simulink model "GridN1"  (R2021a)
settings: Solver=VariableStepAuto  StartTime=0.0  StopTime=1  FixedStep=1e-10  RelTol=1e-3
libraries: spsDistributedParametersLineLib x45, spsThreePhaseSeriesRLCLoadLib x20, spsThreePhaseVIMeasurementLib x3, spsGroundLib x1, spsThreePhaseSourceLib x1, spsSeriesRLCBranchLib x1, spspowerguiLib x1
settings Model: Creator=miair  LastModifiedBy=Admin
settings SolverCC: AlgebraicLoopSolver=TrustRegion
settings DataIOCC: ReturnWorkspaceOutputs=off
settings DebuggingCC: SFMachineParentedDataDiag=warning  ArithmeticOperatorsInVariantConditions=warning
settings SFSimCC: SimUseLocalCustomCode=off  CustomCodeUndefinedFunction=UseInterfaceOnly
settings RTWCC: RTWUseLocalCustomCode=off
settings CodeAppCC: StateflowObjectComments=on
settings SimscapeCC: SimscapeNormalizeSystem=off

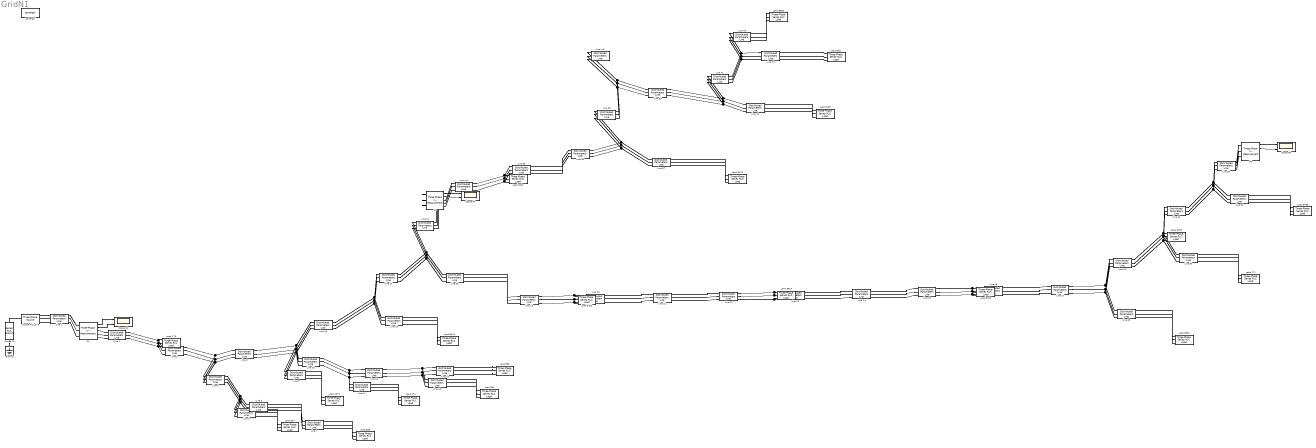
== system GridN1 ==
  Ground : spsGroundLib/Ground  LConnTagsString=a
  Line 1 : spsDistributedParametersLineLib/Distributed Parameters Line  Phases=3  Length=0.01  Frequency=50  Resistance=[0.476003738225748 0.351747138225748 0.351747138225748;0.351747138225748 0.476003738225748 0.351747138225748;0.351747138225748 0.351747138225748 0.476003738225748]  Inductance=[0.000705954362986426 0.000459934243504405 0.000459934243504405;0.000459934243504405 0.000705954362986426 0.000459934243504405;0.000459934243504405 0.000459934243504405 0.000705954362986426]  Capacitance=[5.7561313269996e-07 -1.37543883484145e-07 -1.37543912800485e-07;-1.37543883484145e-07 5.75613027339387e-07 -1.37543875208088e-07;-1.37543912800485e-07 -1.37543875208088e-07 5.75613005057695e-07]  x1=[0.0135819851168218 6580.60780006136 6580.6182267289;314.159265358979 314.159265358979 314.159265358979;-0.926204081652274 -0.816756558113271 -2.38755380781111]  x2=[0.0137023481415946 6580.57590971446 6580.58635696497;314.159265358979 314.159265358979 314.159265358979;-0.934430302579672 -0.816757783153402 -2.38755503539598]  x3=[0.0128763749933069 332.939719946223 332.945796056873;314.159265358979 314.159265358979 314.159265358979;-2.07623123292733 -0.796255794413397 -2.36710494899868]  x4=[0.0127279522499466 375.758691230381 375.75302064917;314.159265358979 314.159265358979 314.159265358979;1.03880908557987 -0.834961314041496 -2.40571318285691]  x5=2.2104317621921e-07  V1=[0.01488 9985 9985;314.2 314.2 314.2;0.4891 -0.0989 -1.67]  V2=[0.01499 9985 9985;314.2 314.2 314.2;0.4801 -0.0989 -1.67]  I1=[0.01357 505.2 505.2;314.2 314.2 314.2;-0.7953 -0.07837 -1.649]  I2=[0.01346 570.2 570.2;314.2 314.2 314.2;2.317 -0.1171 -1.688]  nHarmo=1  Measurements=None  Decoupling=off  VsMag0=0  VrMag0=0  VsAngle0=0  VrAngle0=0  IsMag0=0  IrMag0=0  IsAngle0=0  IrAngle0=0
      settings: SourceProductBaseCode=PS
  Line 10 : spsDistributedParametersLineLib/Distributed Parameters Line  Phases=3  Length=0.16  Frequency=50  Resistance=[0.646656091154803 0.0486237908083191 0.0486712220507153;0.0486237908083191 0.646561225344642 0.0486237934466192;0.0486712220507153 0.0486237934466192 0.646656091154803]  Inductance=[0.00282448912315926 0.00133270803418135 0.00132951476746136;0.00133270803418135 0.00282479813276775 0.00133799988507366;0.00132951476746136 0.00133799988507366 0.00282448912315926]  Capacitance=[7.89543174552926e-09 -1.85986777702161e-09 -1.7901190036642e-09;-1.85986777702161e-09 7.82540023894543e-09 -1.8957321828871e-09;-1.7901190036642e-09 -1.8957321828871e-09 7.91264394645417e-09]  x1=[85.9944639712659 6546.93050475178 6546.44352092211;314.159265358979 314.159265358979 314.159265358979;0.297132510613398 -0.901407935041179 -2.47234114362476]  x2=[85.9964448785897 6546.65446589105 6546.16802554073;314.159265358979 314.159265358979 314.159265358979;0.297142047123019 -0.901418200609058 -2.47235127057814]  x3=[0.0804619526636368 14.5654071899657 14.6911796185752;314.159265358979 314.159265358979 314.159265358979;0.235078954953871 -0.835037872721124 -2.40660973507596]  x4=[0.0702350961721193 18.8073119716894 18.934319702301;314.159265358979 314.159265358979 314.159265358979;0.367987664701655 -0.952972217807643 -2.52350664948334]  x5=7.66635634017784e-07  V1=[130.5 9934 9933;314.2 314.2 314.2;1.015 -0.1836 -1.754]  V2=[130.5 9933 9933;314.2 314.2 314.2;1.015 -0.1836 -1.754]  I1=[0.1221 22.1 22.29;314.2 314.2 314.2;0.9534 -0.1172 -1.689]  I2=[0.1066 28.54 28.73;314.2 314.2 314.2;1.086 -0.2351 -1.806]  nHarmo=1  Measurements=None  Decoupling=off  VsMag0=0  VrMag0=0  VsAngle0=0  VrAngle0=0  IsMag0=0  IrMag0=0  IsAngle0=0  IrAngle0=0
      settings: SourceProductBaseCode=PS
  Line 11 : spsDistributedParametersLineLib/Distributed Parameters Line  Phases=3  Length=0.16  Frequency=50  Resistance=[0.646656091154803 0.0486237908083191 0.0486712220507153;0.0486237908083191 0.646561225344642 0.0486237934466192;0.0486712220507153 0.0486237934466192 0.646656091154803]  Inductance=[0.00282448912315926 0.00133270803418135 0.00132951476746136;0.00133270803418135 0.00282479813276775 0.00133799988507366;0.00132951476746136 0.00133799988507366 0.00282448912315926]  Capacitance=[7.89543174552926e-09 -1.85986777702161e-09 -1.7901190036642e-09;-1.85986777702161e-09 7.82540023894543e-09 -1.8957321828871e-09;-1.7901190036642e-09 -1.8957321828871e-09 7.91264394645417e-09]  x1=[85.9964448785897 6546.65446589105 6546.16802554073;314.159265358979 314.159265358979 314.159265358979;0.297142047123019 -0.901418200609058 -2.47235127057814]  x2=[85.9976584945911 6546.47413610085 6545.98803986244;314.159265358979 314.159265358979 314.159265358979;0.297148477688424 -0.901424241770337 -2.47235721789357]  x3=[0.0785355624578365 15.3056638554528 15.4318437577526;314.159265358979 314.159265358979 314.159265358979;0.259013030174006 -0.858371763028016 -2.42967864630558]  x4=[0.0719518400150709 18.0351581181147 18.1620865019816;314.159265358979 314.159265358979 314.159265358979;0.338516704500895 -0.938129134970429 -2.50878862058241]  x5=7.66635634017784e-07  V1=[130.5 9933 9933;314.2 314.2 314.2;1.015 -0.1836 -1.754]  V2=[130.5 9933 9933;314.2 314.2 314.2;1.015 -0.1836 -1.755]  I1=[0.1192 23.22 23.42;314.2 314.2 314.2;0.9773 -0.1405 -1.712]  I2=[0.1092 27.37 27.56;314.2 314.2 314.2;1.057 -0.2203 -1.791]  nHarmo=1  Measurements=None  Decoupling=off  VsMag0=0  VrMag0=0  VsAngle0=0  VrAngle0=0  IsMag0=0  IrMag0=0  IsAngle0=0  IrAngle0=0
      settings: SourceProductBaseCode=PS
  Line 12 : spsDistributedParametersLineLib/Distributed Parameters Line  Phases=3  Length=0.18  Frequency=50  Resistance=[0.646656091154803 0.0486237908083191 0.0486712220507153;0.0486237908083191 0.646561225344642 0.0486237934466192;0.0486712220507153 0.0486237934466192 0.646656091154803]  Inductance=[0.00282448912315926 0.00133270803418135 0.00132951476746136;0.00133270803418135 0.00282479813276775 0.00133799988507366;0.00132951476746136 0.00133799988507366 0.00282448912315926]  Capacitance=[7.89543174552926e-09 -1.85986777702161e-09 -1.7901190036642e-09;-1.85986777702161e-09 7.82540023894543e-09 -1.8957321828871e-09;-1.7901190036642e-09 -1.8957321828871e-09 7.91264394645417e-09]  x1=[85.9964448785897 6546.65446589105 6546.16802554073;314.159265358979 314.159265358979 314.159265358979;0.297111941412071 -0.901442117619123 -2.47237521035551]  x2=[85.9972993196457 6546.54637248643 6546.06015563724;314.159265358979 314.159265358979 314.159265358979;0.297115479187386 -0.901446788951277 -2.47237983061846]  x3=[0.0770387830362932 15.9012798359736 16.0277069156014;314.159265358979 314.159265358979 314.159265358979;0.271434826795543 -0.88191367645825 -2.45304200019236]  x4=[0.0733797001123517 17.4185010889173 17.5453298819302;314.159265358979 314.159265358979 314.159265358979;0.323795655893711 -0.919479721591919 -2.49024653991903]  x5=8.62465088270006e-07  V1=[130.5 9933 9933;314.2 314.2 314.2;1.015 -0.1836 -1.755]  V2=[130.5 9933 9933;314.2 314.2 314.2;1.015 -0.1836 -1.755]  I1=[0.1169 24.13 24.32;314.2 314.2 314.2;0.9898 -0.1641 -1.735]  I2=[0.1114 26.43 26.62;314.2 314.2 314.2;1.042 -0.2016 -1.772]  nHarmo=1  Measurements=None  Decoupling=off  VsMag0=0  VrMag0=0  VsAngle0=0  VrAngle0=0  IsMag0=0  IrMag0=0  IsAngle0=0  IrAngle0=0
      settings: SourceProductBaseCode=PS
  Line 13 : spsDistributedParametersLineLib/Distributed Parameters Line  Phases=3  Length=0.53  Frequency=50  Resistance=[0.646656091154803 0.0486237908083191 0.0486712220507153;0.0486237908083191 0.646561225344642 0.0486237934466192;0.0486712220507153 0.0486237934466192 0.646656091154803]  Inductance=[0.00282448912315926 0.00133270803418135 0.00132951476746136;0.00133270803418135 0.00282479813276775 0.00133799988507366;0.00132951476746136 0.00133799988507366 0.00282448912315926]  Capacitance=[7.89543174552926e-09 -1.85986777702161e-09 -1.7901190036642e-09;-1.85986777702161e-09 7.82540023894543e-09 -1.8957321828871e-09;-1.7901190036642e-09 -1.8957321828871e-09 7.91264394645417e-09]  x1=[85.9972993196455 6546.54637248643 6546.06015563724;314.159265358979 314.159265358979 314.159265358979;0.296588629245806 -0.901865336627409 -2.47279877672234]  x2=[85.999109686468 6546.2820331029 6545.79632491974;314.159265358979 314.159265358979 314.159265358979;0.296597976971236 -0.901874451699163 -2.47280775550619]  x3=[0.0766475627213019 16.0457568642052 16.1721358047216;314.159265358979 314.159265358979 314.159265358979;0.278553064422003 -0.884195825609553 -2.45528139945166]  x4=[0.0737204509155215 17.2589219147414 17.3856160487695;314.159265358979 314.159265358979 314.159265358979;0.3145362068788 -0.918913142041838 -2.4897144121643]  x5=2.53948053768391e-06  V1=[130.5 9933 9933;314.2 314.2 314.2;1.015 -0.184 -1.755]  V2=[130.5 9933 9932;314.2 314.2 314.2;1.015 -0.184 -1.755]  I1=[0.1163 24.35 24.54;314.2 314.2 314.2;0.9969 -0.1663 -1.737]  I2=[0.1119 26.19 26.38;314.2 314.2 314.2;1.033 -0.2011 -1.772]  nHarmo=1  Measurements=None  Decoupling=off  VsMag0=0  VrMag0=0  VsAngle0=0  VrAngle0=0  IsMag0=0  IrMag0=0  IsAngle0=0  IrAngle0=0
      settings: SourceProductBaseCode=PS
  Line 14 : spsDistributedParametersLineLib/Distributed Parameters Line  Phases=3  Length=2.16  Frequency=50  Resistance=[0.646656091154803 0.0486237908083191 0.0486712220507153;0.0486237908083191 0.646561225344642 0.0486237934466192;0.0486712220507153 0.0486237934466192 0.646656091154803]  Inductance=[0.00282448912315926 0.00133270803418135 0.00132951476746136;0.00133270803418135 0.00282479813276775 0.00133799988507366;0.00132951476746136 0.00133799988507366 0.00282448912315926]  Capacitance=[7.89543174552926e-09 -1.85986777702161e-09 -1.7901190036642e-09;-1.85986777702161e-09 7.82540023894543e-09 -1.8957321828871e-09;-1.7901190036642e-09 -1.8957321828871e-09 7.91264394645417e-09]  x1=[85.9972993196455 6546.54637248643 6546.06015563724;314.159265358979 314.159265358979 314.159265358979;0.294135013803574 -0.903814572947683 -2.47474986857757]  x2=[85.9995705439625 6546.29754411503 6545.81188305122;314.159265358979 314.159265358979 314.159265358979;0.29414239813252 -0.90382784404018 -2.47476303451906]  x3=[0.0754794263753424 16.467720066683 16.5937728872859;314.159265358979 314.159265358979 314.159265358979;0.286520713788774 -0.901964753453352 -2.47293834107752]  x4=[0.0747483168592489 16.7703048358143 16.8964299339934;314.159265358979 314.159265358979 314.159265358979;0.298562747055325 -0.908206004743712 -2.47910645537711]  x5=1.03495810592401e-05  V1=[130.5 9933 9933;314.2 314.2 314.2;1.012 -0.186 -1.757]  V2=[130.5 9933 9932;314.2 314.2 314.2;1.012 -0.186 -1.757]  I1=[0.1145 24.99 25.18;314.2 314.2 314.2;1.005 -0.1841 -1.755]  I2=[0.1134 25.45 25.64;314.2 314.2 314.2;1.017 -0.1904 -1.761]  nHarmo=1  Measurements=None  Decoupling=off  VsMag0=0  VrMag0=0  VsAngle0=0  VrAngle0=0  IsMag0=0  IrMag0=0  IsAngle0=0  IrAngle0=0
      settings: SourceProductBaseCode=PS
  Line 15 : spsDistributedParametersLineLib/Distributed Parameters Line  Phases=3  Length=4.06  Frequency=50  Resistance=[0.502970710632245 0.0486237908083191 0.0486712220507153;0.0486237908083191 0.502875844822084 0.0486237934466192;0.0486712220507153 0.0486237934466192 0.502970710632245]  Inductance=[0.00286900545038753 0.00133270803418135 0.00132951476746136;0.00133270803418135 0.00286931445999602 0.00133799988507366;0.00132951476746136 0.00133799988507366 0.00286900545038753]  Capacitance=[8.11484299003193e-09 -1.94249816214699e-09 -1.86930692621136e-09;-1.94249816214699e-09 8.0425699231653e-09 -1.98049571960044e-09;-1.86930692621136e-09 -1.98049571960044e-09 8.13337738722527e-09]  x1=[155.130058091746 6546.90392964469 6546.32991141257;314.159265358979 314.159265358979 314.159265358979;0.274010343197794 -0.899988695828293 -2.47095312062203]  x2=[155.136487397732 6511.09041009802 6510.62379376133;314.159265358979 314.159265358979 314.159265358979;0.272333769665952 -0.903385149921619 -2.47432401319414]  x3=[0.10391403445318 4.32286136277482 4.3539078763867;314.159265358979 314.159265358979 314.159265358979;0.152577548487083 0.302540110540726 -1.29846084646846]  x4=[0.168935784291522 31.8497990242347 31.9649152376635;314.159265358979 314.159265358979 314.159265358979;0.342256765474295 -1.03135915522522 -2.60124142850109]  x5=1.96604952826627e-05  V1=[235.4 9934 9933;314.2 314.2 314.2;0.9921 -0.1821 -1.753]  V2=[235.4 9879 9879;314.2 314.2 314.2;0.9908 -0.1855 -1.756]  I1=[0.1683 6.565 6.576;314.2 314.2 314.2;0.8807 1.024 -0.5817]  I2=[0.2456 48.35 48.5;314.2 314.2 314.2;1.062 -0.3137 -1.883]  nHarmo=1  Measurements=None  Decoupling=off  VsMag0=0  VrMag0=0  VsAngle0=0  VrAngle0=0  IsMag0=0  IrMag0=0  IsAngle0=0  IrAngle0=0
      settings: SourceProductBaseCode=PS
  Line 16 : spsDistributedParametersLineLib/Distributed Parameters Line  Phases=3  Length=0.01  Frequency=50  Resistance=[0.646656091154803 0.0486237908083191 0.0486712220507153;0.0486237908083191 0.646561225344642 0.0486237934466192;0.0486712220507153 0.0486237934466192 0.646656091154803]  Inductance=[0.00282448912315926 0.00133270803418135 0.00132951476746136;0.00133270803418135 0.00282479813276775 0.00133799988507366;0.00132951476746136 0.00133799988507366 0.00282448912315926]  Capacitance=[7.89543174552926e-09 -1.85986777702161e-09 -1.7901190036642e-09;-1.85986777702161e-09 7.82540023894543e-09 -1.8957321828871e-09;-1.7901190036642e-09 -1.8957321828871e-09 7.91264394645417e-09]  x1=[86.3836277831307 6511.11801645557 6510.73918186067;314.159265358979 314.159265358979 314.159265358979;0.296859447111635 -0.904624882143572 -2.4755324376731]  x2=[86.3836330279052 6511.11723795004 6510.73840482828;314.159265358979 314.159265358979 314.159265358979;0.296859474579558 -0.904624908354452 -2.47553246347659]  x3=[0.075755124590947 16.4755952702995 16.6018616731868;314.159265358979 314.159265358979 314.159265358979;0.294122728550855 -0.901862047196781 -2.4727919470391]  x4=[0.075301162455798 16.6643113475344 16.7906304355618;314.159265358979 314.159265358979 314.159265358979;0.299597594398029 -0.907368346005886 -2.47825404656015]  x5=4.79147271261115e-08  V1=[131.1 9879 9879;314.2 314.2 314.2;1.016 -0.1868 -1.758]  V2=[131.1 9879 9879;314.2 314.2 314.2;1.016 -0.1868 -1.758]  I1=[0.115 25 25.19;314.2 314.2 314.2;1.013 -0.184 -1.755]  I2=[0.1143 25.29 25.48;314.2 314.2 314.2;1.019 -0.1895 -1.76]  nHarmo=1  Measurements=None  Decoupling=off  VsMag0=0  VrMag0=0  VsAngle0=0  VrAngle0=0  IsMag0=0  IrMag0=0  IsAngle0=0  IrAngle0=0
      settings: SourceProductBaseCode=PS
  Line 17 : spsDistributedParametersLineLib/Distributed Parameters Line  Phases=3  Length=0.35  Frequency=50  Resistance=[0.646656091154803 0.0486237908083191 0.0486712220507153;0.0486237908083191 0.646561225344642 0.0486237934466192;0.0486712220507153 0.0486237934466192 0.646656091154803]  Inductance=[0.00282448912315926 0.00133270803418135 0.00132951476746136;0.00133270803418135 0.00282479813276775 0.00133799988507366;0.00132951476746136 0.00133799988507366 0.00282448912315926]  Capacitance=[7.89543174552926e-09 -1.85986777702161e-09 -1.7901190036642e-09;-1.85986777702161e-09 7.82540023894543e-09 -1.8957321828871e-09;-1.7901190036642e-09 -1.8957321828871e-09 7.91264394645417e-09]  x1=[86.3836277831307 6511.11801645557 6510.73918186067;314.159265358979 314.159265358979 314.159265358979;0.296347650025526 -0.905031471314672 -2.4759394138883]  x2=[86.4097152949425 6507.31425320866 6506.94452871459;314.159265358979 314.159265358979 314.159265358979;0.296462312233359 -0.905281202958687 -2.4761870329915]  x3=[0.109465414980559 4.31753359742384 4.35145979089518;314.159265358979 314.159265358979 314.159265358979;0.0135914404706076 0.296780704754496 -1.30398448333316]  x4=[0.0551442407666985 31.8173296486231 31.9338693613861;314.159265358979 314.159265358979 314.159265358979;0.882642018156363 -1.03228675249212 -2.60219232773787]  x5=1.6770154494139e-06  V1=[131.1 9879 9879;314.2 314.2 314.2;1.015 -0.1872 -1.758]  V2=[131.2 9874 9873;314.2 314.2 314.2;1.015 -0.1874 -1.758]  I1=[0.1764 6.557 6.572;314.2 314.2 314.2;0.7506 1.018 -0.5873]  I2=[0.07492 48.3 48.46;314.2 314.2 314.2;1.678 -0.3147 -1.884]  nHarmo=1  Measurements=None  Decoupling=off  VsMag0=0  VrMag0=0  VsAngle0=0  VrAngle0=0  IsMag0=0  IrMag0=0  IsAngle0=0  IrAngle0=0
      settings: SourceProductBaseCode=PS
  Line 18 : spsDistributedParametersLineLib/Distributed Parameters Line  Phases=3  Length=0.26  Frequency=50  Resistance=[0.646656091154803 0.0486237908083191 0.0486712220507153;0.0486237908083191 0.646561225344642 0.0486237934466192;0.0486712220507153 0.0486237934466192 0.646656091154803]  Inductance=[0.00282448912315926 0.00133270803418135 0.00132951476746136;0.00133270803418135 0.00282479813276775 0.00133799988507366;0.00132951476746136 0.00133799988507366 0.00282448912315926]  Capacitance=[7.89543174552926e-09 -1.85986777702161e-09 -1.7901190036642e-09;-1.85986777702161e-09 7.82540023894543e-09 -1.8957321828871e-09;-1.7901190036642e-09 -1.8957321828871e-09 7.91264394645417e-09]  x1=[86.4097152949424 6507.31425320866 6506.94452871459;314.159265358979 314.159265358979 314.159265358979;0.296597787932625 -0.905173576413396 -2.47607930399336]  x2=[86.4164234767737 6506.31319209991 6505.94386622124;314.159265358979 314.159265358979 314.159265358979;0.296676077842439 -0.90529675193356 -2.47620177288688]  x3=[0.0940058289360008 10.0710803597759 10.1963204188777;314.159265358979 314.159265358979 314.159265358979;0.220423677789878 -0.911182921321596 -2.48235367189124]  x4=[0.0577970860777915 23.0375917576632 23.1647009597948;314.159265358979 314.159265358979 314.159265358979;0.420279554992001 -0.902858499466097 -2.47362985744283]  x5=1.2457829052789e-06  V1=[131.2 9874 9873;314.2 314.2 314.2;1.016 -0.1873 -1.758]  V2=[131.2 9872 9872;314.2 314.2 314.2;1.016 -0.1874 -1.758]  I1=[0.1427 15.28 15.47;314.2 314.2 314.2;0.9392 -0.1933 -1.765]  I2=[0.08773 34.96 35.15;314.2 314.2 314.2;1.14 -0.185 -1.756]  nHarmo=1  Measurements=None  Decoupling=off  VsMag0=0  VrMag0=0  VsAngle0=0  VrAngle0=0  IsMag0=0  IrMag0=0  IsAngle0=0  IrAngle0=0
      settings: SourceProductBaseCode=PS
  Line 19 : spsDistributedParametersLineLib/Distributed Parameters Line  Phases=3  Length=0.03  Frequency=50  Resistance=[0.476003738225748 0.351747138225748 0.351747138225748;0.351747138225748 0.476003738225748 0.351747138225748;0.351747138225748 0.351747138225748 0.476003738225748]  Inductance=[0.000705954362986426 0.000459934243504405 0.000459934243504405;0.000459934243504405 0.000705954362986426 0.000459934243504405;0.000459934243504405 0.000459934243504405 0.000705954362986426]  Capacitance=[5.7561313269996e-07 -1.37543883484145e-07 -1.37543912800485e-07;-1.37543883484145e-07 5.75613027339387e-07 -1.37543875208088e-07;-1.37543912800485e-07 -1.37543875208088e-07 5.75613005057695e-07]  x1=[1.80349077964358 6506.96689280743 6507.23152701917;314.159265358979 314.159265358979 314.159265358979;0.568507403599857 -0.823462772990433 -2.39421460640899]  x2=[1.80349908463451 6506.94280065842 6507.20743625873;314.159265358979 314.159265358979 314.159265358979;0.568466669705737 -0.823465104058031 -2.39421693847239]  x3=[0.0240219359496491 343.799843304301 343.813477118347;314.159265358979 314.159265358979 314.159265358979;0.492004045456063 -0.823628998476846 -2.39438530592288]  x4=[0.0251371408204683 356.767166807137 356.781970901396;314.159265358979 314.159265358979 314.159265358979;0.641366971008245 -0.823427454004275 -2.39417497717186]  x5=6.63129528657629e-07  V1=[2.826 9873 9874;314.2 314.2 314.2;1.332 -0.1056 -1.676]  V2=[2.826 9873 9874;314.2 314.2 314.2;1.332 -0.1056 -1.676]  I1=[0.03756 521.7 521.7;314.2 314.2 314.2;1.259 -0.1058 -1.677]  I2=[0.03945 541.3 541.4;314.2 314.2 314.2;1.402 -0.1056 -1.676]  nHarmo=1  Measurements=None  Decoupling=off  VsMag0=0  VrMag0=0  VsAngle0=0  VrAngle0=0  IsMag0=0  IrMag0=0  IsAngle0=0  IrAngle0=0
      settings: SourceProductBaseCode=PS
  Line 2 : spsDistributedParametersLineLib/Distributed Parameters Line  Phases=3  Length=0.67  Frequency=50  Resistance=[0.502970710632245 0.0486237908083191 0.0486712220507153;0.0486237908083191 0.502875844822084 0.0486237934466192;0.0486712220507153 0.0486237934466192 0.502970710632245]  Inductance=[0.00286900545038753 0.00133270803418135 0.00132951476746136;0.00133270803418135 0.00286931445999602 0.00133799988507366;0.00132951476746136 0.00133799988507366 0.00286900545038753]  Capacitance=[8.11484299003193e-09 -1.94249816214699e-09 -1.86930692621136e-09;-1.94249816214699e-09 8.0425699231653e-09 -1.98049571960044e-09;-1.86930692621136e-09 -1.98049571960044e-09 8.13337738722527e-09]  x1=[155.130864966467 6579.86288650135 6579.19403824536;314.159265358979 314.159265358979 314.159265358979;0.280572916473346 -0.892956956254344 -2.46393908894624]  x2=[155.129993894483 6571.12588097019 6570.48183439309;314.159265358979 314.159265358979 314.159265358979;0.280210089543806 -0.893696316191029 -2.46467257592617]  x3=[0.0936269338507397 8.28080195745267 8.1875967056366;314.159265358979 314.159265358979 314.159265358979;0.126927443731738 1.27624388214372 -0.306383861829034]  x4=[0.180082285305984 38.7443835177047 38.8603787264615;314.159265358979 314.159265358979 314.159265358979;0.359177992222435 -1.07116495488925 -2.64099140895834]  x5=3.24446597029163e-06  V1=[235.4 9984 9983;314.2 314.2 314.2;0.9985 -0.1751 -1.746]  V2=[235.4 9971 9970;314.2 314.2 314.2;0.9982 -0.1758 -1.747]  I1=[0.1527 12.59 12.4;314.2 314.2 314.2;0.8579 1.995 0.4132]  I2=[0.2625 58.81 58.96;314.2 314.2 314.2;1.079 -0.3535 -1.923]  nHarmo=1  Measurements=None  Decoupling=off  VsMag0=0  VrMag0=0  VsAngle0=0  VrAngle0=0  IsMag0=0  IrMag0=0  IsAngle0=0  IrAngle0=0
      settings: SourceProductBaseCode=PS
  Line 20 : spsDistributedParametersLineLib/Distributed Parameters Line  Phases=3  Length=0.06  Frequency=50  Resistance=[0.476003738225748 0.351747138225748 0.351747138225748;0.351747138225748 0.476003738225748 0.351747138225748;0.351747138225748 0.351747138225748 0.476003738225748]  Inductance=[0.000705954362986426 0.000459934243504405 0.000459934243504405;0.000459934243504405 0.000705954362986426 0.000459934243504405;0.000459934243504405 0.000459934243504405 0.000705954362986426]  Capacitance=[5.7561313269996e-07 -1.37543883484145e-07 -1.37543912800485e-07;-1.37543883484145e-07 5.75613027339387e-07 -1.37543875208088e-07;-1.37543912800485e-07 -1.37543875208088e-07 5.75613005057695e-07]  x1=[1.80349908463435 6506.94280065843 6507.20743625873;314.159265358979 314.159265358979 314.159265358979;0.568258341420157 -0.823589942694024 -2.39434177709874]  x2=[1.80351546829951 6506.90345923597 6507.16809797319;314.159265358979 314.159265358979 314.159265358979;0.568177174345155 -0.823594380959789 -2.39434621735615]  x3=[0.0240130059935537 344.689458476285 344.70313048417;314.159265358979 314.159265358979 314.159265358979;0.491956343910604 -0.824953446673106 -2.39570974436397]  x4=[0.0251275086274899 355.769214247355 355.783979573751;314.159265358979 314.159265358979 314.159265358979;0.640683073045103 -0.822519085690189 -2.39326659996042]  x5=1.32625905731526e-06  V1=[2.826 9873 9874;314.2 314.2 314.2;1.332 -0.1057 -1.676]  V2=[2.826 9873 9874;314.2 314.2 314.2;1.332 -0.1057 -1.677]  I1=[0.03754 523 523;314.2 314.2 314.2;1.259 -0.1071 -1.678]  I2=[0.03944 539.8 539.9;314.2 314.2 314.2;1.401 -0.1047 -1.675]  nHarmo=1  Measurements=None  Decoupling=off  VsMag0=0  VrMag0=0  VsAngle0=0  VrAngle0=0  IsMag0=0  IrMag0=0  IsAngle0=0  IrAngle0=0
      settings: SourceProductBaseCode=PS
  Line 21 : spsDistributedParametersLineLib/Distributed Parameters Line  Phases=3  Length=0.2  Frequency=50  Resistance=[0.646656091154803 0.0486237908083191 0.0486712220507153;0.0486237908083191 0.646561225344642 0.0486237934466192;0.0486712220507153 0.0486237934466192 0.646656091154803]  Inductance=[0.00282448912315926 0.00133270803418135 0.00132951476746136;0.00133270803418135 0.00282479813276775 0.00133799988507366;0.00132951476746136 0.00133799988507366 0.00282448912315926]  Capacitance=[7.89543174552926e-09 -1.85986777702161e-09 -1.7901190036642e-09;-1.85986777702161e-09 7.82540023894543e-09 -1.8957321828871e-09;-1.7901190036642e-09 -1.8957321828871e-09 7.91264394645417e-09]  x1=[86.4156775370292 6506.24976374386 6505.88045131294;314.159265358979 314.159265358979 314.159265358979;0.296757442469757 -0.905231770339363 -2.47613672584176]  x2=[86.4198873770657 6505.62270406743 6505.25347886743;314.159265358979 314.159265358979 314.159265358979;0.296811157398845 -0.905318825738908 -2.47622331895673]  x3=[0.0915214048129825 11.0184276621565 11.1439055827763;314.159265358979 314.159265358979 314.159265358979;0.237528372241948 -0.939888068634841 -2.51068855775993]  x4=[0.0599840015892358 22.0976245780948 22.2245410295841;314.159265358979 314.159265358979 314.159265358979;0.38688459691695 -0.888198292322438 -2.45905890793362]  x5=9.5829454252223e-07  V1=[131.2 9872 9872;314.2 314.2 314.2;1.016 -0.1874 -1.758]  V2=[131.2 9871 9871;314.2 314.2 314.2;1.016 -0.1875 -1.758]  I1=[0.1389 16.72 16.91;314.2 314.2 314.2;0.9563 -0.222 -1.793]  I2=[0.09104 33.53 33.72;314.2 314.2 314.2;1.106 -0.1703 -1.741]  nHarmo=1  Measurements=None  Decoupling=off  VsMag0=0  VrMag0=0  VsAngle0=0  VrAngle0=0  IsMag0=0  IrMag0=0  IsAngle0=0  IrAngle0=0
      settings: SourceProductBaseCode=PS
  Line 22 : spsDistributedParametersLineLib/Distributed Parameters Line  Phases=3  Length=0.05  Frequency=50  Resistance=[0.476003738225748 0.351747138225748 0.351747138225748;0.351747138225748 0.476003738225748 0.351747138225748;0.351747138225748 0.351747138225748 0.476003738225748]  Inductance=[0.000705954362986426 0.000459934243504405 0.000459934243504405;0.000459934243504405 0.000705954362986426 0.000459934243504405;0.000459934243504405 0.000459934243504405 0.000705954362986426]  Capacitance=[5.7561313269996e-07 -1.37543883484145e-07 -1.37543912800485e-07;-1.37543883484145e-07 5.75613027339387e-07 -1.37543875208088e-07;-1.37543912800485e-07 -1.37543875208088e-07 5.75613005057695e-07]  x1=[1.81872127937186 6506.27610314953 6506.5412101485;314.159265358979 314.159265358979 314.159265358979;0.572739489358775 -0.823639824767842 -2.39439120314015]  x2=[1.81873407318244 6506.24299562844 6506.50810513395;314.159265358979 314.159265358979 314.159265358979;0.572673891127853 -0.823643443820417 -2.39439482381432]  x3=[0.0242231513539572 344.670879322376 344.68458384404;314.159265358979 314.159265358979 314.159265358979;0.498933104195823 -0.824739694137653 -2.39549543281646]  x4=[0.02532942018017 355.751316792513 355.766100937454;314.159265358979 314.159265358979 314.159265358979;0.642913048433806 -0.822782616536565 -2.39352977372954]  x5=1.10521588109605e-06  V1=[2.85 9872 9873;314.2 314.2 314.2;1.336 -0.1058 -1.677]  V2=[2.85 9872 9873;314.2 314.2 314.2;1.336 -0.1058 -1.677]  I1=[0.03787 523 523;314.2 314.2 314.2;1.265 -0.1069 -1.678]  I2=[0.03975 539.8 539.8;314.2 314.2 314.2;1.403 -0.1049 -1.676]  nHarmo=1  Measurements=None  Decoupling=off  VsMag0=0  VrMag0=0  VsAngle0=0  VrAngle0=0  IsMag0=0  IrMag0=0  IsAngle0=0  IrAngle0=0
      settings: SourceProductBaseCode=PS
  Line 23 : spsDistributedParametersLineLib/Distributed Parameters Line  Phases=3  Length=0.05  Frequency=50  Resistance=[0.476003738225748 0.351747138225748 0.351747138225748;0.351747138225748 0.476003738225748 0.351747138225748;0.351747138225748 0.351747138225748 0.476003738225748]  Inductance=[0.000705954362986426 0.000459934243504405 0.000459934243504405;0.000459934243504405 0.000705954362986426 0.000459934243504405;0.000459934243504405 0.000459934243504405 0.000705954362986426]  Capacitance=[5.7561313269996e-07 -1.37543883484145e-07 -1.37543912800485e-07;-1.37543883484145e-07 5.75613027339387e-07 -1.37543875208088e-07;-1.37543912800485e-07 -1.37543875208088e-07 5.75613005057695e-07]  x1=[1.81873407318247 6506.24299562844 6506.50810513395;314.159265358979 314.159265358979 314.159265358979;0.572673891127767 -0.823643443820417 -2.39439482381432]  x2=[1.81874665516727 6506.21722820899 6506.48234052024;314.159265358979 314.159265358979 314.159265358979;0.572608571318828 -0.823646869350555 -2.39439825096607]  x3=[0.0242227990722459 345.612328664751 345.626073424913;314.159265358979 314.159265358979 314.159265358979;0.499219322631955 -0.825850429726011 -2.39660615929487]  x4=[0.0253288933872046 354.807869311172 354.822616843042;314.159265358979 314.159265358979 314.159265358979;0.642511794453256 -0.82170242285628 -2.39244957127083]  x5=1.10521588109605e-06  V1=[2.85 9872 9873;314.2 314.2 314.2;1.336 -0.1058 -1.677]  V2=[2.85 9872 9873;314.2 314.2 314.2;1.336 -0.1058 -1.677]  I1=[0.03787 524.4 524.4;314.2 314.2 314.2;1.265 -0.108 -1.679]  I2=[0.03975 538.4 538.4;314.2 314.2 314.2;1.403 -0.1038 -1.675]  nHarmo=1  Measurements=None  Decoupling=off  VsMag0=0  VrMag0=0  VsAngle0=0  VrAngle0=0  IsMag0=0  IrMag0=0  IsAngle0=0  IrAngle0=0
      settings: SourceProductBaseCode=PS
  Line 24 : spsDistributedParametersLineLib/Distributed Parameters Line  Phases=3  Length=0.07  Frequency=50  Resistance=[0.646656091154803 0.0486237908083191 0.0486712220507153;0.0486237908083191 0.646561225344642 0.0486237934466192;0.0486712220507153 0.0486237934466192 0.646656091154803]  Inductance=[0.00282448912315926 0.00133270803418135 0.00132951476746136;0.00133270803418135 0.00282479813276775 0.00133799988507366;0.00132951476746136 0.00133799988507366 0.00282448912315926]  Capacitance=[7.89543174552926e-09 -1.85986777702161e-09 -1.7901190036642e-09;-1.85986777702161e-09 7.82540023894543e-09 -1.8957321828871e-09;-1.7901190036642e-09 -1.8957321828871e-09 7.91264394645417e-09]  x1=[86.4192070770427 6505.56383378223 6505.19462260516;314.159265358979 314.159265358979 314.159265358979;0.296997423813308 -0.905170409868426 -2.47607475819285]  x2=[86.4203532262805 6505.39397464631 6505.02472042426;314.159265358979 314.159265358979 314.159265358979;0.297013900777833 -0.90519809985593 -2.47610231497634]  x3=[0.0890553814813472 11.9746385535509 12.1002847514108;314.159265358979 314.159265358979 314.159265358979;0.255140561932488 -0.96277099212005 -2.53331866081606]  x4=[0.06224838038178 21.1652048696928 21.2919280563146;314.159265358979 314.159265358979 314.159265358979;0.356790003617149 -0.872681161888096 -2.44364213900161]  x5=3.3540308988278e-07  V1=[131.2 9871 9871;314.2 314.2 314.2;1.016 -0.1873 -1.758]  V2=[131.2 9871 9870;314.2 314.2 314.2;1.016 -0.1873 -1.758]  I1=[0.1352 18.17 18.36;314.2 314.2 314.2;0.9739 -0.2449 -1.815]  I2=[0.09448 32.11 32.31;314.2 314.2 314.2;1.076 -0.1548 -1.726]  nHarmo=1  Measurements=None  Decoupling=off  VsMag0=0  VrMag0=0  VsAngle0=0  VrAngle0=0  IsMag0=0  IrMag0=0  IsAngle0=0  IrAngle0=0
      settings: SourceProductBaseCode=PS
  Line 25 : spsDistributedParametersLineLib/Distributed Parameters Line  Phases=3  Length=0.28  Frequency=50  Resistance=[0.476003738225748 0.351747138225748 0.351747138225748;0.351747138225748 0.476003738225748 0.351747138225748;0.351747138225748 0.351747138225748 0.476003738225748]  Inductance=[0.000705954362986426 0.000459934243504405 0.000459934243504405;0.000459934243504405 0.000705954362986426 0.000459934243504405;0.000459934243504405 0.000459934243504405 0.000705954362986426]  Capacitance=[5.7561313269996e-07 -1.37543883484145e-07 -1.37543912800485e-07;-1.37543883484145e-07 5.75613027339387e-07 -1.37543875208088e-07;-1.37543912800485e-07 -1.37543875208088e-07 5.75613005057695e-07]  x1=[1.8230209208266 6506.04728504326 6506.31246540836;314.159265358979 314.159265358979 314.159265358979;0.572485854467426 -0.824631656746514 -2.39538290476063]  x2=[1.8230863268609 6505.89775727232 6506.16295295788;314.159265358979 314.159265358979 314.159265358979;0.572128374768087 -0.824649547749504 -2.39540080477212]  x3=[0.0242137936707559 345.201325872334 345.215060458315;314.159265358979 314.159265358979 314.159265358979;0.499985173074447 -0.826625035667704 -2.39738059969799]  x4=[0.0253117804131848 354.382690207975 354.397421274766;314.159265358979 314.159265358979 314.159265358979;0.639582549208556 -0.823858187108396 -2.39460524216789]  x5=6.18920893413787e-06  V1=[2.856 9872 9872;314.2 314.2 314.2;1.336 -0.1068 -1.678]  V2=[2.856 9872 9872;314.2 314.2 314.2;1.335 -0.1068 -1.678]  I1=[0.03786 523.8 523.8;314.2 314.2 314.2;1.266 -0.1088 -1.68]  I2=[0.03972 537.7 537.7;314.2 314.2 314.2;1.4 -0.106 -1.677]  nHarmo=1  Measurements=None  Decoupling=off  VsMag0=0  VrMag0=0  VsAngle0=0  VrAngle0=0  IsMag0=0  IrMag0=0  IsAngle0=0  IrAngle0=0
      settings: SourceProductBaseCode=PS
  Line 26 : spsDistributedParametersLineLib/Distributed Parameters Line  Phases=3  Length=0.28  Frequency=50  Resistance=[0.476003738225748 0.351747138225748 0.351747138225748;0.351747138225748 0.476003738225748 0.351747138225748;0.351747138225748 0.351747138225748 0.476003738225748]  Inductance=[0.000705954362986426 0.000459934243504405 0.000459934243504405;0.000459934243504405 0.000705954362986426 0.000459934243504405;0.000459934243504405 0.000459934243504405 0.000705954362986426]  Capacitance=[5.7561313269996e-07 -1.37543883484145e-07 -1.37543912800485e-07;-1.37543883484145e-07 5.75613027339387e-07 -1.37543875208088e-07;-1.37543912800485e-07 -1.37543875208088e-07 5.75613005057695e-07]  x1=[1.82308632686094 6505.89775727232 6506.16295295788;314.159265358979 314.159265358979 314.159265358979;0.572128374768 -0.824649547749504 -2.39540080477212]  x2=[1.82314506449276 6505.80768545556 6506.07289888839;314.159265358979 314.159265358979 314.159265358979;0.571779641739294 -0.82466414612788 -2.39541541215957]  x3=[0.0242118510820579 346.700996752661 346.714795023725;314.159265358979 314.159265358979 314.159265358979;0.501603433603007 -0.827563523571792 -2.39831907914342]  x4=[0.0253088324522552 352.871323867619 352.885995815209;314.159265358979 314.159265358979 314.159265358979;0.637346398018359 -0.822956511028876 -2.39370355757977]  x5=6.18920893413787e-06  V1=[2.856 9872 9872;314.2 314.2 314.2;1.335 -0.1068 -1.678]  V2=[2.856 9871 9872;314.2 314.2 314.2;1.335 -0.1068 -1.678]  I1=[0.03786 526.1 526.1;314.2 314.2 314.2;1.267 -0.1097 -1.68]  I2=[0.03971 535.4 535.5;314.2 314.2 314.2;1.398 -0.1051 -1.676]  nHarmo=1  Measurements=None  Decoupling=off  VsMag0=0  VrMag0=0  VsAngle0=0  VrAngle0=0  IsMag0=0  IrMag0=0  IsAngle0=0  IrAngle0=0
      settings: SourceProductBaseCode=PS
  Line 27 : spsDistributedParametersLineLib/Distributed Parameters Line  Phases=3  Length=1.36  Frequency=50  Resistance=[0.646656091154803 0.0486237908083191 0.0486712220507153;0.0486237908083191 0.646561225344642 0.0486237934466192;0.0486712220507153 0.0486237934466192 0.646656091154803]  Inductance=[0.00282448912315926 0.00133270803418135 0.00132951476746136;0.00133270803418135 0.00282479813276775 0.00133799988507366;0.00132951476746136 0.00133799988507366 0.00282448912315926]  Capacitance=[7.89543174552926e-09 -1.85986777702161e-09 -1.7901190036642e-09;-1.85986777702161e-09 7.82540023894543e-09 -1.8957321828871e-09;-1.7901190036642e-09 -1.8957321828871e-09 7.91264394645417e-09]  x1=[86.41769096282 6505.15439208593 6504.78521075975;314.159265358979 314.159265358979 314.159265358979;0.295026529136134 -0.906773237020136 -2.47767893780055]  x2=[86.4328195511921 6503.01773940534 6502.64772259314;314.159265358979 314.159265358979 314.159265358979;0.29524317366834 -0.907150728180629 -2.47805473425713]  x3=[0.0846368417931134 13.4543777295203 13.5798836296032;314.159265358979 314.159265358979 314.159265358979;0.264119123882452 -0.951540255530786 -2.52221363055765]  x4=[0.0664789790041574 19.6203863280902 19.7464623844457;314.159265358979 314.159265358979 314.159265358979;0.332298413527271 -0.877769655149948 -2.44874836970492]  x5=6.51640288915116e-06  V1=[131.2 9870 9870;314.2 314.2 314.2;1.014 -0.1889 -1.76]  V2=[131.2 9867 9867;314.2 314.2 314.2;1.014 -0.1893 -1.76]  I1=[0.1285 20.41 20.61;314.2 314.2 314.2;0.9829 -0.2337 -1.804]  I2=[0.1009 29.77 29.96;314.2 314.2 314.2;1.051 -0.1599 -1.731]  nHarmo=1  Measurements=None  Decoupling=off  VsMag0=0  VrMag0=0  VsAngle0=0  VrAngle0=0  IsMag0=0  IrMag0=0  IsAngle0=0  IrAngle0=0
      settings: SourceProductBaseCode=PS
  Line 28 : spsDistributedParametersLineLib/Distributed Parameters Line  Phases=3  Length=1.36  Frequency=50  Resistance=[0.646656091154803 0.0486237908083191 0.0486712220507153;0.0486237908083191 0.646561225344642 0.0486237934466192;0.0486712220507153 0.0486237934466192 0.646656091154803]  Inductance=[0.00282448912315926 0.00133270803418135 0.00132951476746136;0.00133270803418135 0.00282479813276775 0.00133799988507366;0.00132951476746136 0.00133799988507366 0.00282448912315926]  Capacitance=[7.89543174552926e-09 -1.85986777702161e-09 -1.7901190036642e-09;-1.85986777702161e-09 7.82540023894543e-09 -1.8957321828871e-09;-1.7901190036642e-09 -1.8957321828871e-09 7.91264394645417e-09]  x1=[86.432819551192 6503.01773940534 6502.64772259314;314.159265358979 314.159265358979 314.159265358979;0.29524317366834 -0.907150728180629 -2.47805473425713]  x2=[86.4358465140095 6502.60313253252 6502.23393095589;314.159265358979 314.159265358979 314.159265358979;0.295257166475471 -0.907166619093573 -2.47807041738444]  x3=[0.0764327310054961 16.1480008970677 16.2736603621684;314.159265358979 314.159265358979 314.159265358979;0.282432237923772 -0.897517036086079 -2.46851468013547]  x4=[0.0746231852296247 16.9002921608203 17.0261517412317;314.159265358979 314.159265358979 314.159265358979;0.306306472739271 -0.917962093622172 -2.48878123583803]  x5=6.51640288915116e-06  V1=[131.2 9867 9867;314.2 314.2 314.2;1.014 -0.1893 -1.76]  V2=[131.2 9867 9866;314.2 314.2 314.2;1.014 -0.1893 -1.76]  I1=[0.116 24.5 24.69;314.2 314.2 314.2;1.001 -0.1797 -1.751]  I2=[0.1133 25.64 25.83;314.2 314.2 314.2;1.025 -0.2001 -1.771]  nHarmo=1  Measurements=None  Decoupling=off  VsMag0=0  VrMag0=0  VsAngle0=0  VrAngle0=0  IsMag0=0  IrMag0=0  IsAngle0=0  IrAngle0=0
      settings: SourceProductBaseCode=PS
  Line 29 : spsDistributedParametersLineLib/Distributed Parameters Line  Phases=3  Length=0.17  Frequency=50  Resistance=[0.646656091154803 0.0486237908083191 0.0486712220507153;0.0486237908083191 0.646561225344642 0.0486237934466192;0.0486712220507153 0.0486237934466192 0.646656091154803]  Inductance=[0.00282448912315926 0.00133270803418135 0.00132951476746136;0.00133270803418135 0.00282479813276775 0.00133799988507366;0.00132951476746136 0.00133799988507366 0.00282448912315926]  Capacitance=[7.89543174552926e-09 -1.85986777702161e-09 -1.7901190036642e-09;-1.85986777702161e-09 7.82540023894543e-09 -1.8957321828871e-09;-1.7901190036642e-09 -1.8957321828871e-09 7.91264394645417e-09]  x1=[86.432819551192 6503.01773940534 6502.64772259314;314.159265358979 314.159265358979 314.159265358979;0.297034463469724 -0.905727666081779 -2.47663031750393]  x2=[86.434284429277 6502.80026347489 6502.43003551985;314.159265358979 314.159265358979 314.159265358979;0.29706002975242 -0.905772436283474 -2.47667489798959]  x3=[0.0837639229819949 13.8516275904661 13.9774558111502;314.159265358979 314.159265358979 314.159265358979;0.279314022527542 -0.958642201946851 -2.52920580776062]  x4=[0.0673964365811018 19.2734917918798 19.3997898951826;314.159265358979 314.159265358979 314.159265358979;0.318800689564801 -0.86792033126489 -2.43897167655951]  x5=8.14550361143895e-07  V1=[131.2 9867 9867;314.2 314.2 314.2;1.016 -0.1879 -1.759]  V2=[131.2 9867 9867;314.2 314.2 314.2;1.016 -0.1879 -1.759]  I1=[0.1272 21.02 21.21;314.2 314.2 314.2;0.9981 -0.2408 -1.811]  I2=[0.1023 29.24 29.44;314.2 314.2 314.2;1.038 -0.1501 -1.721]  nHarmo=1  Measurements=None  Decoupling=off  VsMag0=0  VrMag0=0  VsAngle0=0  VrAngle0=0  IsMag0=0  IrMag0=0  IsAngle0=0  IrAngle0=0
      settings: SourceProductBaseCode=PS
  Line 3 : spsDistributedParametersLineLib/Distributed Parameters Line  Phases=3  Length=0.91  Frequency=50  Resistance=[0.502970710632245 0.0486237908083191 0.0486712220507153;0.0486237908083191 0.502875844822084 0.0486237934466192;0.0486712220507153 0.0486237934466192 0.502970710632245]  Inductance=[0.00286900545038753 0.00133270803418135 0.00132951476746136;0.00133270803418135 0.00286931445999602 0.00133799988507366;0.00132951476746136 0.00133799988507366 0.00286900545038753]  Capacitance=[8.11484299003193e-09 -1.94249816214699e-09 -1.86930692621136e-09;-1.94249816214699e-09 8.0425699231653e-09 -1.98049571960044e-09;-1.86930692621136e-09 -1.98049571960044e-09 8.13337738722527e-09]  x1=[155.129993894483 6571.12588097019 6570.48183439309;314.159265358979 314.159265358979 314.159265358979;0.27984497466176 -0.893992012210619 -2.46496860471872]  x2=[155.128790736444 6559.40096916411 6558.79015535965;314.159265358979 314.159265358979 314.159265358979;0.279356759579792 -0.894989960274266 -2.4659586226253]  x3=[0.093989526604838 8.07452294892549 7.98284003890752;314.159265358979 314.159265358979 314.159265358979;0.128185047972175 1.26260829622213 -0.320479826476611]  x4=[0.179654012055719 38.4703653562676 38.5861620676527;314.159265358979 314.159265358979 314.159265358979;0.357545367096607 -1.07072456038996 -2.64055255496118]  x5=4.40666273576923e-06  V1=[235.4 9971 9970;314.2 314.2 314.2;0.9978 -0.1761 -1.747]  V2=[235.4 9953 9952;314.2 314.2 314.2;0.9974 -0.1771 -1.748]  I1=[0.1532 12.28 12.09;314.2 314.2 314.2;0.8591 1.981 0.3991]  I2=[0.2618 58.4 58.55;314.2 314.2 314.2;1.077 -0.3531 -1.922]  nHarmo=1  Measurements=None  Decoupling=off  VsMag0=0  VrMag0=0  VsAngle0=0  VrAngle0=0  IsMag0=0  IrMag0=0  IsAngle0=0  IrAngle0=0
      settings: SourceProductBaseCode=PS
  Line 30 : spsDistributedParametersLineLib/Distributed Parameters Line  Phases=3  Length=1.32  Frequency=50  Resistance=[0.476003738225748 0.351747138225748 0.351747138225748;0.351747138225748 0.476003738225748 0.351747138225748;0.351747138225748 0.351747138225748 0.476003738225748]  Inductance=[0.000705954362986426 0.000459934243504405 0.000459934243504405;0.000459934243504405 0.000705954362986426 0.000459934243504405;0.000459934243504405 0.000459934243504405 0.000705954362986426]  Capacitance=[5.7561313269996e-07 -1.37543883484145e-07 -1.37543912800485e-07;-1.37543883484145e-07 5.75613027339387e-07 -1.37543875208088e-07;-1.37543912800485e-07 -1.37543875208088e-07 5.75613005057695e-07]  x1=[1.88476507349602 6503.45237684542 6503.71811596765;314.159265358979 314.159265358979 314.159265358979;0.586463226737287 -0.829414169659759 -2.40016353616277]  x2=[1.88484425879095 6503.42176602541 6503.68750388167;314.159265358979 314.159265358979 314.159265358979;0.586366221924231 -0.829440517346566 -2.40018988384582]  x3=[0.0252226472009313 347.240423534723 347.254585494499;314.159265358979 314.159265358979 314.159265358979;0.577248791667439 -0.834091143927947 -2.40484050993932]  x4=[0.0252226331623234 348.436027567525 348.450238381863;314.159265358979 314.159265358979 314.159265358979;0.586365704192308 -0.830275128015271 -2.40102449457919]  x5=2.91776992609357e-05  V1=[2.953 9868 9868;314.2 314.2 314.2;1.347 -0.1116 -1.682]  V2=[2.953 9868 9868;314.2 314.2 314.2;1.347 -0.1116 -1.682]  I1=[0.03951 526.9 526.9;314.2 314.2 314.2;1.338 -0.1162 -1.687]  I2=[0.03951 528.7 528.7;314.2 314.2 314.2;1.347 -0.1124 -1.683]  nHarmo=1  Measurements=None  Decoupling=off  VsMag0=0  VrMag0=0  VsAngle0=0  VrAngle0=0  IsMag0=0  IrMag0=0  IsAngle0=0  IrAngle0=0
      settings: SourceProductBaseCode=PS
  Line 31 : spsDistributedParametersLineLib/Distributed Parameters Line  Phases=3  Length=1.33  Frequency=50  Resistance=[0.646656091154803 0.0486237908083191 0.0486712220507153;0.0486237908083191 0.646561225344642 0.0486237934466192;0.0486712220507153 0.0486237934466192 0.646656091154803]  Inductance=[0.00282448912315926 0.00133270803418135 0.00132951476746136;0.00133270803418135 0.00282479813276775 0.00133799988507366;0.00132951476746136 0.00133799988507366 0.00282448912315926]  Capacitance=[7.89543174552926e-09 -1.85986777702161e-09 -1.7901190036642e-09;-1.85986777702161e-09 7.82540023894543e-09 -1.8957321828871e-09;-1.7901190036642e-09 -1.8957321828871e-09 7.91264394645417e-09]  x1=[86.434284429277 6502.80026347489 6502.43003551985;314.159265358979 314.159265358979 314.159265358979;0.295313898517459 -0.907159622867227 -2.47806340507674]  x2=[86.4401556149764 6502.2054539875 6501.83660108807;314.159265358979 314.159265358979 314.159265358979;0.295330123010291 -0.90719502897051 -2.47809857528239]  x3=[0.0769981213379446 15.9222854212303 16.0478760007592;314.159265358979 314.159265358979 314.159265358979;0.26915353281551 -0.896411518028236 -2.46747220265232]  x4=[0.0741040018327553 17.1259027642474 17.2518149799855;314.159265358979 314.159265358979 314.159265358979;0.320471149933708 -0.918721840790863 -2.48948662662382]  x5=6.37265870777283e-06  V1=[131.2 9867 9867;314.2 314.2 314.2;1.014 -0.1893 -1.76]  V2=[131.2 9866 9866;314.2 314.2 314.2;1.014 -0.1893 -1.76]  I1=[0.1169 24.16 24.35;314.2 314.2 314.2;0.9881 -0.1786 -1.75]  I2=[0.1125 25.99 26.18;314.2 314.2 314.2;1.039 -0.2009 -1.772]  nHarmo=1  Measurements=None  Decoupling=off  VsMag0=0  VrMag0=0  VsAngle0=0  VrAngle0=0  IsMag0=0  IrMag0=0  IsAngle0=0  IrAngle0=0
      settings: SourceProductBaseCode=PS
  Line 32 : spsDistributedParametersLineLib/Distributed Parameters Line  Phases=3  Length=0.18  Frequency=50  Resistance=[0.646656091154803 0.0486237908083191 0.0486712220507153;0.0486237908083191 0.646561225344642 0.0486237934466192;0.0486712220507153 0.0486237934466192 0.646656091154803]  Inductance=[0.00282448912315926 0.00133270803418135 0.00132951476746136;0.00133270803418135 0.00282479813276775 0.00133799988507366;0.00132951476746136 0.00133799988507366 0.00282448912315926]  Capacitance=[7.89543174552926e-09 -1.85986777702161e-09 -1.7901190036642e-09;-1.85986777702161e-09 7.82540023894543e-09 -1.8957321828871e-09;-1.7901190036642e-09 -1.8957321828871e-09 7.91264394645417e-09]  x1=[86.4401556149765 6502.2054539875 6501.83660108807;314.159265358979 314.159265358979 314.159265358979;0.29706120138978 -0.905819800891789 -2.47672203808392]  x2=[86.440761419296 6502.1159911893 6501.7473078187;314.159265358979 314.159265358979 314.159265358979;0.2970643389286 -0.905822839340956 -2.47672502976343]  x3=[0.0770313773387684 15.9436280558103 16.0695320312976;314.159265358979 314.159265358979 314.159265358979;0.279661585097967 -0.887718182633114 -2.45877227272522]  x4=[0.0741346195948001 17.1492471367742 17.2754899875772;314.159265358979 314.159265358979 314.159265358979;0.314867712096174 -0.922859352536945 -2.49362949229038]  x5=8.62465088270006e-07  V1=[131.2 9866 9866;314.2 314.2 314.2;1.016 -0.188 -1.759]  V2=[131.2 9866 9866;314.2 314.2 314.2;1.016 -0.188 -1.759]  I1=[0.1169 24.19 24.38;314.2 314.2 314.2;0.9986 -0.1699 -1.741]  I2=[0.1125 26.02 26.21;314.2 314.2 314.2;1.034 -0.205 -1.776]  nHarmo=1  Measurements=None  Decoupling=off  VsMag0=0  VrMag0=0  VsAngle0=0  VrAngle0=0  IsMag0=0  IrMag0=0  IsAngle0=0  IrAngle0=0
      settings: SourceProductBaseCode=PS
  Line 33 : spsDistributedParametersLineLib/Distributed Parameters Line  Phases=3  Length=4.6  Frequency=50  Resistance=[0.646656091154803 0.0486237908083191 0.0486712220507153;0.0486237908083191 0.646561225344642 0.0486237934466192;0.0486712220507153 0.0486237934466192 0.646656091154803]  Inductance=[0.00282448912315926 0.00133270803418135 0.00132951476746136;0.00133270803418135 0.00282479813276775 0.00133799988507366;0.00132951476746136 0.00133799988507366 0.00282448912315926]  Capacitance=[7.89543174552926e-09 -1.85986777702161e-09 -1.7901190036642e-09;-1.85986777702161e-09 7.82540023894543e-09 -1.8957321828871e-09;-1.7901190036642e-09 -1.8957321828871e-09 7.91264394645417e-09]  x1=[86.4401556149765 6502.2054539875 6501.83660108807;314.159265358979 314.159265358979 314.159265358979;0.290407839270354 -0.911105460116089 -2.48201272888152]  x2=[86.4422278878468 6502.30383281083 6501.93516169722;314.159265358979 314.159265358979 314.159265358979;0.290397500712476 -0.911124710406228 -2.48203214204633]  x3=[0.0754104044481364 16.4610405218583 16.5858774411566;314.159265358979 314.159265358979 314.159265358979;0.283478356353729 -0.916615997721408 -2.48752858440473]  x4=[0.0754104057963133 16.4610409568714 16.5858778835961;314.159265358979 314.159265358979 314.159265358979;0.290397500713952 -0.911124710406212 -2.4820321420463]  x5=2.20407744780113e-05  V1=[131.2 9866 9866;314.2 314.2 314.2;1.009 -0.1933 -1.764]  V2=[131.2 9866 9866;314.2 314.2 314.2;1.009 -0.1933 -1.764]  I1=[0.1145 24.98 25.17;314.2 314.2 314.2;1.002 -0.1988 -1.77]  I2=[0.1145 24.98 25.17;314.2 314.2 314.2;1.009 -0.1933 -1.764]  nHarmo=1  Measurements=None  Decoupling=off  VsMag0=0  VrMag0=0  VsAngle0=0  VrAngle0=0  IsMag0=0  IrMag0=0  IsAngle0=0  IrAngle0=0
      settings: SourceProductBaseCode=PS
  Line 34 : spsDistributedParametersLineLib/Distributed Parameters Line  Phases=3  Length=0.35  Frequency=50  Resistance=[0.646656091154803 0.0486237908083191 0.0486712220507153;0.0486237908083191 0.646561225344642 0.0486237934466192;0.0486712220507153 0.0486237934466192 0.646656091154803]  Inductance=[0.00282448912315926 0.00133270803418135 0.00132951476746136;0.00133270803418135 0.00282479813276775 0.00133799988507366;0.00132951476746136 0.00133799988507366 0.00282448912315926]  Capacitance=[7.89543174552926e-09 -1.85986777702161e-09 -1.7901190036642e-09;-1.85986777702161e-09 7.82540023894543e-09 -1.8957321828871e-09;-1.7901190036642e-09 -1.8957321828871e-09 7.91264394645417e-09]  x1=[86.4097152949424 6507.31425320866 6506.94452871459;314.159265358979 314.159265358979 314.159265358979;0.296462312233361 -0.905281202958687 -2.4761870329915]  x2=[86.4267405969679 6504.85680112977 6504.49564242131;314.159265358979 314.159265358979 314.159265358979;0.29647170369327 -0.905365018864096 -2.47626968272231]  x3=[0.0900277394201515 9.01248144668122 9.12570593737069;314.159265358979 314.159265358979 314.159265358979;0.034084926138278 -0.434159664050808 -2.01302599681262]  x4=[0.0682493821005929 25.4035353687568 25.5184947922303;314.159265358979 314.159265358979 314.159265358979;0.645050997400067 -1.06734334411212 -2.63697988152164]  x5=1.6770154494139e-06  V1=[131.2 9874 9873;314.2 314.2 314.2;1.015 -0.1874 -1.758]  V2=[131.2 9870 9870;314.2 314.2 314.2;1.016 -0.1875 -1.758]  I1=[0.1469 13.66 13.83;314.2 314.2 314.2;0.7735 0.2853 -1.297]  I2=[0.09356 38.57 38.72;314.2 314.2 314.2;1.4 -0.3498 -1.918]  nHarmo=1  Measurements=None  Decoupling=off  VsMag0=0  VrMag0=0  VsAngle0=0  VrAngle0=0  IsMag0=0  IrMag0=0  IsAngle0=0  IrAngle0=0
      settings: SourceProductBaseCode=PS
  Line 35 : spsDistributedParametersLineLib/Distributed Parameters Line  Phases=3  Length=0.09  Frequency=50  Resistance=[0.646656091154803 0.0486237908083191 0.0486712220507153;0.0486237908083191 0.646561225344642 0.0486237934466192;0.0486712220507153 0.0486237934466192 0.646656091154803]  Inductance=[0.00282448912315926 0.00133270803418135 0.00132951476746136;0.00133270803418135 0.00282479813276775 0.00133799988507366;0.00132951476746136 0.00133799988507366 0.00282448912315926]  Capacitance=[7.89543174552926e-09 -1.85986777702161e-09 -1.7901190036642e-09;-1.85986777702161e-09 7.82540023894543e-09 -1.8957321828871e-09;-1.7901190036642e-09 -1.8957321828871e-09 7.91264394645417e-09]  x1=[86.4267405969802 6504.85680112907 6504.49564242061;314.159265358979 314.159265358979 314.159265358979;0.296863077935591 -0.905054097733279 -2.47595846561659]  x2=[86.4303546910819 6504.44912994283 6504.08993188391;314.159265358979 314.159265358979 314.159265358979;0.296875042150563 -0.905068254462186 -2.47597226484656]  x3=[0.0913139578614685 11.3452175081703 11.4878591719375;314.159265358979 314.159265358979 314.159265358979;0.106868942822149 -0.671829519329756 -2.24580038527554]  x4=[0.0638286806680737 22.2212767209969 22.3259029374083;314.159265358979 314.159265358979 314.159265358979;0.57028621646809 -1.02341878131962 -2.59370685950682]  x5=4.31232544135003e-07  V1=[131.2 9870 9870;314.2 314.2 314.2;1.016 -0.1872 -1.758]  V2=[131.2 9869 9869;314.2 314.2 314.2;1.016 -0.1872 -1.758]  I1=[0.1477 17.22 17.41;314.2 314.2 314.2;0.7511 0.04794 -1.529]  I2=[0.09504 33.73 33.89;314.2 314.2 314.2;1.435 -0.3065 -1.875]  nHarmo=1  Measurements=None  Decoupling=off  VsMag0=0  VrMag0=0  VsAngle0=0  VrAngle0=0  IsMag0=0  IrMag0=0  IsAngle0=0  IrAngle0=0
      settings: SourceProductBaseCode=PS
  Line 36 : spsDistributedParametersLineLib/Distributed Parameters Line  Phases=3  Length=0.32  Frequency=50  Resistance=[0.502970710632245 0.0486237908083191 0.0486712220507153;0.0486237908083191 0.502875844822084 0.0486237934466192;0.0486712220507153 0.0486237934466192 0.502970710632245]  Inductance=[0.00286900545038753 0.00133270803418135 0.00132951476746136;0.00133270803418135 0.00286931445999602 0.00133799988507366;0.00132951476746136 0.00133799988507366 0.00286900545038753]  Capacitance=[8.11484299003193e-09 -1.94249816214699e-09 -1.86930692621136e-09;-1.94249816214699e-09 8.0425699231653e-09 -1.98049571960044e-09;-1.86930692621136e-09 -1.98049571960044e-09 8.13337738722527e-09]  x1=[155.112035685048 6504.42138667982 6503.97426550552;314.159265358979 314.159265358979 314.159265358979;0.277962980689356 -0.89912494265493 -2.47005497791888]  x2=[155.113411964264 6503.213014458 6502.77203779073;314.159265358979 314.159265358979 314.159265358979;0.277926071667147 -0.899197520280986 -2.4701262761427]  x3=[0.127692552150037 11.3509489070479 11.493279398651;314.159265358979 314.159265358979 314.159265358979;0.235428963071931 -0.665856634488038 -2.23992149237215]  x4=[0.144578967086316 22.2240972665342 22.3284904761638;314.159265358979 314.159265358979 314.159265358979;0.315033534924227 -1.01781534342222 -2.58809221385254]  x5=1.54959568730346e-06  V1=[235.4 9869 9869;314.2 314.2 314.2;0.9965 -0.1813 -1.752]  V2=[235.4 9867 9867;314.2 314.2 314.2;0.9964 -0.1813 -1.752]  I1=[0.2015 17.22 17.42;314.2 314.2 314.2;0.8937 0.0539 -1.523]  I2=[0.2135 33.73 33.89;314.2 314.2 314.2;1.093 -0.3009 -1.869]  nHarmo=1  Measurements=None  Decoupling=off  VsMag0=0  VrMag0=0  VsAngle0=0  VrAngle0=0  IsMag0=0  IrMag0=0  IsAngle0=0  IrAngle0=0
      settings: SourceProductBaseCode=PS
  Line 37 : spsDistributedParametersLineLib/Distributed Parameters Line  Phases=3  Length=0.06  Frequency=50  Resistance=[0.646656091154803 0.0486237908083191 0.0486712220507153;0.0486237908083191 0.646561225344642 0.0486237934466192;0.0486712220507153 0.0486237934466192 0.646656091154803]  Inductance=[0.00282448912315926 0.00133270803418135 0.00132951476746136;0.00133270803418135 0.00282479813276775 0.00133799988507366;0.00132951476746136 0.00133799988507366 0.00282448912315926]  Capacitance=[7.89543174552926e-09 -1.85986777702161e-09 -1.7901190036642e-09;-1.85986777702161e-09 7.82540023894543e-09 -1.8957321828871e-09;-1.7901190036642e-09 -1.8957321828871e-09 7.91264394645417e-09]  x1=[86.4445732020567 6503.24081543001 6502.88774640087;314.159265358979 314.159265358979 314.159265358979;0.296904037901544 -0.90510495465063 -2.4760076515085]  x2=[86.4447743828698 6503.21095600256 6502.85794335749;314.159265358979 314.159265358979 314.159265358979;0.296905089514867 -0.905105960926195 -2.4760086421387]  x3=[0.077040905448562 15.94841485843 16.0744120147427;314.159265358979 314.159265358979 314.159265358979;0.279697364934227 -0.886855213534287 -2.45790966072538]  x4=[0.074141014727175 17.1544561745712 17.2807969454168;314.159265358979 314.159265358979 314.159265358979;0.314692775744537 -0.922141723354478 -2.49291235396919]  x5=2.87488362756669e-07  V1=[131.2 9868 9867;314.2 314.2 314.2;1.016 -0.1873 -1.758]  V2=[131.2 9867 9867;314.2 314.2 314.2;1.016 -0.1873 -1.758]  I1=[0.117 24.2 24.39;314.2 314.2 314.2;0.9987 -0.169 -1.74]  I2=[0.1126 26.03 26.22;314.2 314.2 314.2;1.034 -0.2043 -1.775]  nHarmo=1  Measurements=None  Decoupling=off  VsMag0=0  VrMag0=0  VsAngle0=0  VrAngle0=0  IsMag0=0  IrMag0=0  IsAngle0=0  IrAngle0=0
      settings: SourceProductBaseCode=PS
  Line 38 : spsDistributedParametersLineLib/Distributed Parameters Line  Phases=3  Length=0.2  Frequency=50  Resistance=[0.502970710632245 0.0486237908083191 0.0486712220507153;0.0486237908083191 0.502875844822084 0.0486237934466192;0.0486712220507153 0.0486237934466192 0.502970710632245]  Inductance=[0.00286900545038753 0.00133270803418135 0.00132951476746136;0.00133270803418135 0.00286931445999602 0.00133799988507366;0.00132951476746136 0.00133799988507366 0.00286900545038753]  Capacitance=[8.11484299003193e-09 -1.94249816214699e-09 -1.86930692621136e-09;-1.94249816214699e-09 8.0425699231653e-09 -1.98049571960044e-09;-1.86930692621136e-09 -1.98049571960044e-09 8.13337738722527e-09]  x1=[155.113411964264 6503.213014458 6502.77203779073;314.159265358979 314.159265358979 314.159265358979;0.278108629108169 -0.899049672271191 -2.46997826174642]  x2=[155.114369867267 6502.54024451109 6502.10290765923;314.159265358979 314.159265358979 314.159265358979;0.278087936805599 -0.899090062130136 -2.47001790283232]  x3=[0.128731316465425 11.8772911518526 12.0210237983715;314.159265358979 314.159265358979 314.159265358979;0.236603059943992 -0.700812310683344 -2.27430241661663]  x4=[0.143548933292522 21.5928321435659 21.6972397812282;314.159265358979 314.159265358979 314.159265358979;0.315019590166148 -1.00781296452093 -2.57812982491454]  x5=9.68497304564665e-07  V1=[235.4 9867 9867;314.2 314.2 314.2;0.9966 -0.1812 -1.752]  V2=[235.4 9866 9866;314.2 314.2 314.2;0.9966 -0.1812 -1.752]  I1=[0.203 18.02 18.22;314.2 314.2 314.2;0.8953 0.01886 -1.558]  I2=[0.2119 32.77 32.93;314.2 314.2 314.2;1.093 -0.2909 -1.859]  nHarmo=1  Measurements=None  Decoupling=off  VsMag0=0  VrMag0=0  VsAngle0=0  VrAngle0=0  IsMag0=0  IrMag0=0  IsAngle0=0  IrAngle0=0
      settings: SourceProductBaseCode=PS
  Line 39 : spsDistributedParametersLineLib/Distributed Parameters Line  Phases=3  Length=0.29  Frequency=50  Resistance=[0.646656091154803 0.0486237908083191 0.0486712220507153;0.0486237908083191 0.646561225344642 0.0486237934466192;0.0486712220507153 0.0486237934466192 0.646656091154803]  Inductance=[0.00282448912315926 0.00133270803418135 0.00132951476746136;0.00133270803418135 0.00282479813276775 0.00133799988507366;0.00132951476746136 0.00133799988507366 0.00282448912315926]  Capacitance=[7.89543174552926e-09 -1.85986777702161e-09 -1.7901190036642e-09;-1.85986777702161e-09 7.82540023894543e-09 -1.8957321828871e-09;-1.7901190036642e-09 -1.8957321828871e-09 7.91264394645417e-09]  x1=[86.4526795774757 6502.568079258 6502.21863894495;314.159265358979 314.159265358979 314.159265358979;0.296548470204786 -0.905420389221007 -2.4763225988307]  x2=[86.460637697514 6501.39879470093 6501.05157216004;314.159265358979 314.159265358979 314.159265358979;0.296589434136902 -0.905460449862099 -2.47636205009561]  x3=[0.0880285657020348 11.8789773629007 12.0010294069323;314.159265358979 314.159265358979 314.159265358979;0.172684208868044 -0.70674172372119 -2.27980179351552]  x4=[0.0647238626529299 21.5659514626468 21.6925501563607;314.159265358979 314.159265358979 314.159265358979;0.464913657731553 -1.01465204670473 -2.58485588944304]  x5=1.38952708665723e-06  V1=[131.2 9866 9866;314.2 314.2 314.2;1.016 -0.1876 -1.758]  V2=[131.3 9865 9864;314.2 314.2 314.2;1.016 -0.1876 -1.759]  I1=[0.1336 18.02 18.21;314.2 314.2 314.2;0.8916 0.01111 -1.562]  I2=[0.09829 32.72 32.92;314.2 314.2 314.2;1.184 -0.2968 -1.867]  nHarmo=1  Measurements=None  Decoupling=off  VsMag0=0  VrMag0=0  VsAngle0=0  VrAngle0=0  IsMag0=0  IrMag0=0  IsAngle0=0  IrAngle0=0
      settings: SourceProductBaseCode=PS
  Line 4 : spsDistributedParametersLineLib/Distributed Parameters Line  Phases=3  Length=0.53  Frequency=50  Resistance=[0.502970710632245 0.0486237908083191 0.0486712220507153;0.0486237908083191 0.502875844822084 0.0486237934466192;0.0486712220507153 0.0486237934466192 0.502970710632245]  Inductance=[0.00286900545038753 0.00133270803418135 0.00132951476746136;0.00133270803418135 0.00286931445999602 0.00133799988507366;0.00132951476746136 0.00133799988507366 0.00286900545038753]  Capacitance=[8.11484299003193e-09 -1.94249816214699e-09 -1.86930692621136e-09;-1.94249816214699e-09 8.0425699231653e-09 -1.98049571960044e-09;-1.86930692621136e-09 -1.98049571960044e-09 8.13337738722527e-09]  x1=[155.128790736444 6559.40096916411 6558.79015535965;314.159265358979 314.159265358979 314.159265358979;0.279934858143029 -0.894521774909914 -2.46548991037043]  x2=[155.127296808445 6558.13489477757 6557.5269745023;314.159265358979 314.159265358979 314.159265358979;0.279897935233285 -0.894606197622115 -2.46557351717579]  x3=[0.129964705404091 13.1744679889912 13.2992539503531;314.159265358979 314.159265358979 314.159265358979;0.275898869119956 -0.777263367834401 -2.34944330790015]  x4=[0.142098007558931 20.3602967014215 20.4873621998356;314.159265358979 314.159265358979 314.159265358979;0.282818953665896 -0.970900913236732 -2.54133000957622]  x5=2.56651785709636e-06  V1=[235.4 9953 9952;314.2 314.2 314.2;0.998 -0.1767 -1.748]  V2=[235.4 9951 9950;314.2 314.2 314.2;0.9979 -0.1768 -1.748]  I1=[0.1972 19.99 20.18;314.2 314.2 314.2;0.9939 -0.05941 -1.632]  I2=[0.2156 30.89 31.09;314.2 314.2 314.2;1.001 -0.253 -1.823]  nHarmo=1  Measurements=None  Decoupling=off  VsMag0=0  VrMag0=0  VsAngle0=0  VrAngle0=0  IsMag0=0  IrMag0=0  IsAngle0=0  IrAngle0=0
      settings: SourceProductBaseCode=PS
  Line 40 : spsDistributedParametersLineLib/Distributed Parameters Line  Phases=3  Length=0.57  Frequency=50  Resistance=[0.646656091154803 0.0486237908083191 0.0486712220507153;0.0486237908083191 0.646561225344642 0.0486237934466192;0.0486712220507153 0.0486237934466192 0.646656091154803]  Inductance=[0.00282448912315926 0.00133270803418135 0.00132951476746136;0.00133270803418135 0.00282479813276775 0.00133799988507366;0.00132951476746136 0.00133799988507366 0.00282448912315926]  Capacitance=[7.89543174552926e-09 -1.85986777702161e-09 -1.7901190036642e-09;-1.85986777702161e-09 7.82540023894543e-09 -1.8957321828871e-09;-1.7901190036642e-09 -1.8957321828871e-09 7.91264394645417e-09]  x1=[86.4606376975138 6501.39879470093 6501.05157216004;314.159265358979 314.159265358979 314.159265358979;0.296167954183639 -0.905795288003005 -2.47669720697872]  x2=[86.4654376607295 6500.69101910482 6500.3451365362;314.159265358979 314.159265358979 314.159265358979;0.296192789999565 -0.905819402327285 -2.47672095161294]  x3=[0.079268885252194 15.0450983741603 15.1705365449213;314.159265358979 314.159265358979 314.159265358979;0.253763737397384 -0.858003366821134 -2.42932859641373]  x4=[0.0720312440249212 18.0542387687365 18.1805598413731;314.159265358979 314.159265358979 314.159265358979;0.341960662318185 -0.946263952721812 -2.51686646521244]  x5=2.73113944618835e-06  V1=[131.3 9865 9864;314.2 314.2 314.2;1.015 -0.1879 -1.759]  V2=[131.3 9864 9863;314.2 314.2 314.2;1.015 -0.188 -1.759]  I1=[0.1203 22.83 23.02;314.2 314.2 314.2;0.9728 -0.1402 -1.711]  I2=[0.1094 27.39 27.59;314.2 314.2 314.2;1.061 -0.2284 -1.799]  nHarmo=1  Measurements=None  Decoupling=off  VsMag0=0  VrMag0=0  VsAngle0=0  VrAngle0=0  IsMag0=0  IrMag0=0  IsAngle0=0  IrAngle0=0
      settings: SourceProductBaseCode=PS
  Line 41 : spsDistributedParametersLineLib/Distributed Parameters Line  Phases=3  Length=0.17  Frequency=50  Resistance=[0.646656091154803 0.0486237908083191 0.0486712220507153;0.0486237908083191 0.646561225344642 0.0486237934466192;0.0486712220507153 0.0486237934466192 0.646656091154803]  Inductance=[0.00282448912315926 0.00133270803418135 0.00132951476746136;0.00133270803418135 0.00282479813276775 0.00133799988507366;0.00132951476746136 0.00133799988507366 0.00282448912315926]  Capacitance=[7.89543174552926e-09 -1.85986777702161e-09 -1.7901190036642e-09;-1.85986777702161e-09 7.82540023894543e-09 -1.8957321828871e-09;-1.7901190036642e-09 -1.8957321828871e-09 7.91264394645417e-09]  x1=[86.4606376975138 6501.39879470093 6501.05157216004;314.159265358979 314.159265358979 314.159265358979;0.296770068402591 -0.905316947801711 -2.47621841143143]  x2=[86.4638541449269 6500.92363348849 6500.57730973761;314.159265358979 314.159265358979 314.159265358979;0.296786756877513 -0.905333086526081 -2.47623430174033]  x3=[0.084075673296631 13.2519718101953 13.3761048313451;314.159265358979 314.159265358979 314.159265358979;0.207650433487107 -0.781899213115493 -2.35401419946518]  x4=[0.0678512766237418 19.9988389284126 20.1254437722575;314.159265358979 314.159265358979 314.159265358979;0.407010258208202 -0.987163514609156 -2.5575089835751]  x5=8.14550361143895e-07  V1=[131.3 9865 9864;314.2 314.2 314.2;1.016 -0.1875 -1.758]  V2=[131.3 9864 9864;314.2 314.2 314.2;1.016 -0.1875 -1.758]  I1=[0.1276 20.11 20.3;314.2 314.2 314.2;0.9266 -0.06405 -1.636]  I2=[0.103 30.34 30.54;314.2 314.2 314.2;1.126 -0.2693 -1.84]  nHarmo=1  Measurements=None  Decoupling=off  VsMag0=0  VrMag0=0  VsAngle0=0  VrAngle0=0  IsMag0=0  IrMag0=0  IsAngle0=0  IrAngle0=0
      settings: SourceProductBaseCode=PS
  Line 42 : spsDistributedParametersLineLib/Distributed Parameters Line  Phases=3  Length=0.01  Frequency=50  Resistance=[0.502970710632245 0.0486237908083191 0.0486712220507153;0.0486237908083191 0.502875844822084 0.0486237934466192;0.0486712220507153 0.0486237934466192 0.502970710632245]  Inductance=[0.00286900545038753 0.00133270803418135 0.00132951476746136;0.00133270803418135 0.00286931445999602 0.00133799988507366;0.00132951476746136 0.00133799988507366 0.00286900545038753]  Capacitance=[8.11484299003193e-09 -1.94249816214699e-09 -1.86930692621136e-09;-1.94249816214699e-09 8.0425699231653e-09 -1.98049571960044e-09;-1.86930692621136e-09 -1.98049571960044e-09 8.13337738722527e-09]  x1=[155.10798566569 6500.89576606593 6500.46151010739;314.159265358979 314.159265358979 314.159265358979;0.278388569683853 -0.898912174814613 -2.46983888942282]  x2=[155.107970633255 6500.88538586235 6500.45115470842;314.159265358979 314.159265358979 314.159265358979;0.278388279133709 -0.898912786524382 -2.46983949464336]  x3=[0.133451954994775 15.0630146539418 15.1885075262535;314.159265358979 314.159265358979 314.159265358979;0.278177944883755 -0.850416551981628 -2.4217770665702]  x4=[0.138629647760991 18.0747219157518 18.2011369041312;314.159265358979 314.159265358979 314.159265358979;0.278576115922384 -0.939334207125443 -2.5099527552823]  x5=4.84248652282332e-08  V1=[235.4 9864 9864;314.2 314.2 314.2;0.9969 -0.1811 -1.752]  V2=[235.4 9864 9864;314.2 314.2 314.2;0.9969 -0.1811 -1.752]  I1=[0.2026 22.86 23.05;314.2 314.2 314.2;0.9967 -0.1326 -1.704]  I2=[0.2104 27.43 27.62;314.2 314.2 314.2;0.9971 -0.2215 -1.792]  nHarmo=1  Measurements=None  Decoupling=off  VsMag0=0  VrMag0=0  VsAngle0=0  VrAngle0=0  IsMag0=0  IrMag0=0  IsAngle0=0  IrAngle0=0
      settings: SourceProductBaseCode=PS
  Line 43 : spsDistributedParametersLineLib/Distributed Parameters Line  Phases=3  Length=0.41  Frequency=50  Resistance=[0.646656091154803 0.0486237908083191 0.0486712220507153;0.0486237908083191 0.646561225344642 0.0486237934466192;0.0486712220507153 0.0486237934466192 0.646656091154803]  Inductance=[0.00282448912315926 0.00133270803418135 0.00132951476746136;0.00133270803418135 0.00282479813276775 0.00133799988507366;0.00132951476746136 0.00133799988507366 0.00282448912315926]  Capacitance=[7.89543174552926e-09 -1.85986777702161e-09 -1.7901190036642e-09;-1.85986777702161e-09 7.82540023894543e-09 -1.8957321828871e-09;-1.7901190036642e-09 -1.8957321828871e-09 7.91264394645417e-09]  x1=[86.4638541449267 6500.92363348849 6500.57730973761;314.159265358979 314.159265358979 314.159265358979;0.296425488346142 -0.905620090646858 -2.4765215790687]  x2=[86.4681575418714 6500.28671958464 6499.94159941557;314.159265358979 314.159265358979 314.159265358979;0.296447875789302 -0.905641659797723 -2.47654281486432]  x3=[0.0802201700407756 14.6808373137041 14.8061032725131;314.159265358979 314.159265358979 314.159265358979;0.244468909229996 -0.843971350419683 -2.41542721572688]  x4=[0.0711778130693579 18.4408411733892 18.5672516948926;314.159265358979 314.159265358979 314.159265358979;0.354356982855002 -0.955147146478187 -2.525689149842]  x5=1.96450381217057e-06  V1=[131.3 9864 9864;314.2 314.2 314.2;1.015 -0.1878 -1.759]  V2=[131.3 9863 9863;314.2 314.2 314.2;1.015 -0.1878 -1.759]  I1=[0.1218 22.28 22.47;314.2 314.2 314.2;0.9635 -0.1261 -1.698]  I2=[0.1081 27.98 28.17;314.2 314.2 314.2;1.073 -0.2373 -1.808]  nHarmo=1  Measurements=None  Decoupling=off  VsMag0=0  VrMag0=0  VsAngle0=0  VrAngle0=0  IsMag0=0  IrMag0=0  IsAngle0=0  IrAngle0=0
      settings: SourceProductBaseCode=PS
  Line 5 : spsDistributedParametersLineLib/Distributed Parameters Line  Phases=3  Length=0.26  Frequency=50  Resistance=[0.502970710632245 0.0486237908083191 0.0486712220507153;0.0486237908083191 0.502875844822084 0.0486237934466192;0.0486712220507153 0.0486237934466192 0.502970710632245]  Inductance=[0.00286900545038753 0.00133270803418135 0.00132951476746136;0.00133270803418135 0.00286931445999602 0.00133799988507366;0.00132951476746136 0.00133799988507366 0.00286900545038753]  Capacitance=[8.11484299003193e-09 -1.94249816214699e-09 -1.86930692621136e-09;-1.94249816214699e-09 8.0425699231653e-09 -1.98049571960044e-09;-1.86930692621136e-09 -1.98049571960044e-09 8.13337738722527e-09]  x1=[155.127296808445 6558.13489477756 6557.5269745023;314.159265358979 314.159265358979 314.159265358979;0.280308689475585 -0.894273539600076 -2.46524048478417]  x2=[155.126692084046 6557.70642420594 6557.09954044014;314.159265358979 314.159265358979 314.159265358979;0.28029665357467 -0.894298632762098 -2.46526531261485]  x3=[0.13193181370902 14.3468981315348 14.4725137889234;314.159265358979 314.159265358979 314.159265358979;0.279506714745316 -0.81368181127468 -2.38540981915086]  x4=[0.140156397573181 19.1233719489417 19.2504334715739;314.159265358979 314.159265358979 314.159265358979;0.280667971659553 -0.955009225592819 -2.52553206947783]  x5=1.25904649593406e-06  V1=[235.4 9951 9950;314.2 314.2 314.2;0.9983 -0.1764 -1.747]  V2=[235.4 9950 9949;314.2 314.2 314.2;0.9983 -0.1764 -1.747]  I1=[0.2002 21.77 21.96;314.2 314.2 314.2;0.9975 -0.09583 -1.668]  I2=[0.2127 29.02 29.21;314.2 314.2 314.2;0.9987 -0.2372 -1.808]  nHarmo=1  Measurements=None  Decoupling=off  VsMag0=0  VrMag0=0  VsAngle0=0  VrAngle0=0  IsMag0=0  IrMag0=0  IsAngle0=0  IrAngle0=0
      settings: SourceProductBaseCode=PS
  Line 6 : spsDistributedParametersLineLib/Distributed Parameters Line  Phases=3  Length=0.06  Frequency=50  Resistance=[0.502970710632245 0.0486237908083191 0.0486712220507153;0.0486237908083191 0.502875844822084 0.0486237934466192;0.0486712220507153 0.0486237934466192 0.502970710632245]  Inductance=[0.00286900545038753 0.00133270803418135 0.00132951476746136;0.00133270803418135 0.00286931445999602 0.00133799988507366;0.00132951476746136 0.00133799988507366 0.00286900545038753]  Capacitance=[8.11484299003193e-09 -1.94249816214699e-09 -1.86930692621136e-09;-1.94249816214699e-09 8.0425699231653e-09 -1.98049571960044e-09;-1.86930692621136e-09 -1.98049571960044e-09 8.13337738722527e-09]  x1=[155.127296808445 6558.13489477757 6557.5269745023;314.159265358979 314.159265358979 314.159265358979;0.280612951877289 -0.894027126250417 -2.46499379412371]  x2=[155.127258095839 6558.09019272422 6557.48236021371;314.159265358979 314.159265358979 314.159265358979;0.280611569763007 -0.894030858722283 -2.46499749511911]  x3=[0.13409993715582 15.4862779379683 15.6127415315502;314.159265358979 314.159265358979 314.159265358979;0.27830638619761 -0.86837743921496 -2.43958020580895]  x4=[0.138010830473366 17.9184598826928 18.04543053236;314.159265358979 314.159265358979 314.159265358979;0.282762806373692 -0.916266993935843 -2.48705327194926]  x5=2.90549191369399e-07  V1=[235.4 9951 9950;314.2 314.2 314.2;0.9986 -0.1762 -1.747]  V2=[235.4 9951 9950;314.2 314.2 314.2;0.9986 -0.1762 -1.747]  I1=[0.2035 23.5 23.69;314.2 314.2 314.2;0.9963 -0.1505 -1.722]  I2=[0.2094 27.19 27.38;314.2 314.2 314.2;1.001 -0.1984 -1.769]  nHarmo=1  Measurements=None  Decoupling=off  VsMag0=0  VrMag0=0  VsAngle0=0  VrAngle0=0  IsMag0=0  IrMag0=0  IsAngle0=0  IrAngle0=0
      settings: SourceProductBaseCode=PS
  Line 7 : spsDistributedParametersLineLib/Distributed Parameters Line  Phases=3  Length=0.13  Frequency=50  Resistance=[0.476003738225748 0.351747138225748 0.351747138225748;0.351747138225748 0.476003738225748 0.351747138225748;0.351747138225748 0.351747138225748 0.476003738225748]  Inductance=[0.000705954362986426 0.000459934243504405 0.000459934243504405;0.000459934243504405 0.000705954362986426 0.000459934243504405;0.000459934243504405 0.000459934243504405 0.000705954362986426]  Capacitance=[5.7561313269996e-07 -1.37543883484145e-07 -1.37543912800485e-07;-1.37543883484145e-07 5.75613027339387e-07 -1.37543875208088e-07;-1.37543912800485e-07 -1.37543875208088e-07 5.75613005057695e-07]  x1=[0.530928938099513 6558.79397335956 6558.87778771663;314.159265358979 314.159265358979 314.159265358979;0.526592644931679 -0.819081842855484 -2.3898659859676]  x2=[0.530929155375503 6558.769363325 6558.85317736743;314.159265358979 314.159265358979 314.159265358979;0.526591714326717 -0.819082490621436 -2.38986663373351]  x3=[0.0072071338038853 351.681298709417 351.685765556187;314.159265358979 314.159265358979 314.159265358979;0.525693312412009 -0.817950249645295 -2.38873439258525]  x4=[0.00720709744673464 354.112117189535 354.116615099275;314.159265358979 314.159265358979 314.159265358979;0.526587824479364 -0.820745541620102 -2.39152968486051]  x5=2.87356129084973e-06  V1=[0.8308 9952 9952;314.2 314.2 314.2;1.289 -0.1012 -1.672]  V2=[0.8308 9952 9952;314.2 314.2 314.2;1.289 -0.1012 -1.672]  I1=[0.01128 533.6 533.6;314.2 314.2 314.2;1.288 -0.1001 -1.671]  I2=[0.01128 537.3 537.3;314.2 314.2 314.2;1.289 -0.1029 -1.674]  nHarmo=1  Measurements=None  Decoupling=off  VsMag0=0  VrMag0=0  VsAngle0=0  VrAngle0=0  IsMag0=0  IrMag0=0  IsAngle0=0  IrAngle0=0
      settings: SourceProductBaseCode=PS
  Line 8 : spsDistributedParametersLineLib/Distributed Parameters Line  Phases=3  Length=1.19  Frequency=50  Resistance=[0.502970710632245 0.0486237908083191 0.0486712220507153;0.0486237908083191 0.502875844822084 0.0486237934466192;0.0486712220507153 0.0486237934466192 0.502970710632245]  Inductance=[0.00286900545038753 0.00133270803418135 0.00132951476746136;0.00133270803418135 0.00286931445999602 0.00133799988507366;0.00132951476746136 0.00133799988507366 0.00286900545038753]  Capacitance=[8.11484299003193e-09 -1.94249816214699e-09 -1.86930692621136e-09;-1.94249816214699e-09 8.0425699231653e-09 -1.98049571960044e-09;-1.86930692621136e-09 -1.98049571960044e-09 8.13337738722527e-09]  x1=[155.128790736444 6559.40096916411 6558.79015535965;314.159265358979 314.159265358979 314.159265358979;0.278930792217405 -0.895334938963788 -2.46630398954994]  x2=[155.130058091747 6546.90392964469 6546.32991141257;314.159265358979 314.159265358979 314.159265358979;0.278376508662248 -0.896452664260691 -2.46741310964445]  x3=[0.0998886193551142 5.26033741103483 5.21804745306695;314.159265358979 314.159265358979 314.159265358979;0.14329353325028 0.845975389880925 -0.749283699485598]  x4=[0.173523190592822 34.6266687723568 34.7426518113543;314.159265358979 314.159265358979 314.159265358979;0.354991019566268 -1.04687043746066 -2.61670442828504]  x5=5.76255896215976e-06  V1=[235.4 9953 9952;314.2 314.2 314.2;0.997 -0.1775 -1.748]  V2=[235.4 9934 9933;314.2 314.2 314.2;0.9965 -0.1786 -1.75]  I1=[0.1622 7.999 7.888;314.2 314.2 314.2;0.8726 1.566 -0.03018]  I2=[0.2526 52.56 52.72;314.2 314.2 314.2;1.075 -0.3292 -1.898]  nHarmo=1  Measurements=None  Decoupling=off  VsMag0=0  VrMag0=0  VsAngle0=0  VrAngle0=0  IsMag0=0  IrMag0=0  IsAngle0=0  IrAngle0=0
      settings: SourceProductBaseCode=PS
  Line 9 : spsDistributedParametersLineLib/Distributed Parameters Line  Phases=3  Length=0.01  Frequency=50  Resistance=[0.646656091154803 0.0486237908083191 0.0486712220507153;0.0486237908083191 0.646561225344642 0.0486237934466192;0.0486712220507153 0.0486237934466192 0.646656091154803]  Inductance=[0.00282448912315926 0.00133270803418135 0.00132951476746136;0.00133270803418135 0.00282479813276775 0.00133799988507366;0.00132951476746136 0.00133799988507366 0.00282448912315926]  Capacitance=[7.89543174552926e-09 -1.85986777702161e-09 -1.7901190036642e-09;-1.85986777702161e-09 7.82540023894543e-09 -1.8957321828871e-09;-1.7901190036642e-09 -1.8957321828871e-09 7.91264394645417e-09]  x1=[85.9944639712659 6546.93050475178 6546.44352092211;314.159265358979 314.159265358979 314.159265358979;0.297358303445506 -0.901228557465694 -2.47216159529453]  x2=[85.9944850086069 6546.92737219904 6546.44039434132;314.159265358979 314.159265358979 314.159265358979;0.297358415273692 -0.901228662036437 -2.4721616982333]  x3=[0.0761074088210107 16.2825529969671 16.4091600989981;314.159265358979 314.159265358979 314.159265358979;0.286481680895019 -0.889947767669242 -2.46097312460605]  x4=[0.0742769121468062 17.0415257172939 17.1683332254368;314.159265358979 314.159265358979 314.159265358979;0.308487857879357 -0.912018713062322 -2.48286710532459]  x5=4.79147271261115e-08  V1=[130.5 9934 9933;314.2 314.2 314.2;1.016 -0.1834 -1.754]  V2=[130.5 9934 9933;314.2 314.2 314.2;1.016 -0.1834 -1.754]  I1=[0.1155 24.71 24.9;314.2 314.2 314.2;1.005 -0.1721 -1.743]  I2=[0.1127 25.86 26.05;314.2 314.2 314.2;1.027 -0.1942 -1.765]  nHarmo=1  Measurements=None  Decoupling=off  VsMag0=0  VrMag0=0  VsAngle0=0  VrAngle0=0  IsMag0=0  IrMag0=0  IsAngle0=0  IrAngle0=0
      settings: SourceProductBaseCode=PS
  Line im1 : spsDistributedParametersLineLib/Distributed Parameters Line  Phases=3  Length=1e-10  Frequency=50  Resistance=[0.646656091154803 0.0486237908083191 0.0486712220507153;0.0486237908083191 0.646561225344642 0.0486237934466192;0.0486712220507153 0.0486237934466192 0.646656091154803]  Inductance=[0.00282448912315926 0.00133270803418135 0.00132951476746136;0.00133270803418135 0.00282479813276775 0.00133799988507366;0.00132951476746136 0.00133799988507366 0.00282448912315926]  Capacitance=[7.89543174552926e-09 -1.85986777702161e-09 -1.7901190036642e-09;-1.85986777702161e-09 7.82540023894543e-09 -1.8957321828871e-09;-1.7901190036642e-09 -1.8957321828871e-09 7.91264394645417e-09]  x1=[86.4267405969678 6504.85680112977 6504.49564242131;314.159265358979 314.159265358979 314.159265358979;0.296998553634703 -0.904946471188083 -2.47585073661855]  x2=[86.4267405969803 6504.85680112907 6504.49564242061;314.159265358979 314.159265358979 314.159265358979;0.296998553634703 -0.904946471188107 -2.47585073661857]  x3=[0.117549279469566 8.96130431772791 9.10145388971096;314.159265358979 314.159265358979 314.159265358979;-0.192689733867281 -0.435344697785911 -2.01052025062557]  x4=[0.0811737409279993 25.4351908475818 25.5550550479186;314.159265358979 314.159265358979 314.159265358979;1.15378928983742 -1.06529479801762 -2.63619789744182]  x5=4.79147271261115e-16  V1=[131.2 9870 9870;314.2 314.2 314.2;1.016 -0.1871 -1.758]  V2=[131.2 9870 9870;314.2 314.2 314.2;1.016 -0.1871 -1.758]  I1=[0.2398 13.66 13.81;314.2 314.2 314.2;0.8853 0.2938 -1.299]  I2=[0.03832 38.62 38.72;314.2 314.2 314.2;2.429 -0.3515 -1.916]  nHarmo=1  Measurements=None  Decoupling=off  VsMag0=0  VrMag0=0  VsAngle0=0  VrAngle0=0  IsMag0=0  IrMag0=0  IsAngle0=0  IrAngle0=0
      settings: SourceProductBaseCode=PS
  Line im2 : spsDistributedParametersLineLib/Distributed Parameters Line  Phases=3  Length=1e-10  Frequency=50  Resistance=[0.502970710632245 0.0486237908083191 0.0486712220507153;0.0486237908083191 0.502875844822084 0.0486237934466192;0.0486712220507153 0.0486237934466192 0.502970710632245]  Inductance=[0.00286900545038753 0.00133270803418135 0.00132951476746136;0.00133270803418135 0.00286931445999602 0.00133799988507366;0.00132951476746136 0.00133799988507366 0.00286900545038753]  Capacitance=[8.11484299003193e-09 -1.94249816214699e-09 -1.86930692621136e-09;-1.94249816214699e-09 8.0425699231653e-09 -1.98049571960044e-09;-1.86930692621136e-09 -1.98049571960044e-09 8.13337738722527e-09]  x1=[155.114369867267 6502.54024451109 6502.10290765923;314.159265358979 314.159265358979 314.159265358979;0.27839219920715 -0.898843648780601 -2.46977121217199]  x2=[155.114369867271 6502.54024451109 6502.10290765924;314.159265358979 314.159265358979 314.159265358979;0.27839219920717 -0.898843648780602 -2.46977121217199]  x3=[0.159141072420341 16.5488825345724 16.7303999232311;314.159265358979 314.159265358979 314.159265358979;0.166604413822897 -0.906350980763965 -2.47266105911576]  x4=[0.104531955109972 16.5761036480317 16.6368283670546;314.159265358979 314.159265358979 314.159265358979;0.439509609067233 -0.891095804672514 -2.46653376361345]  x5=4.84248652282332e-16  V1=[235.4 9866 9866;314.2 314.2 314.2;0.9969 -0.181 -1.752]  V2=[235.4 9866 9866;314.2 314.2 314.2;0.9969 -0.181 -1.752]  I1=[0.2274 25 25.29;314.2 314.2 314.2;0.9378 -0.1792 -1.751]  I2=[0.1889 25.23 25.34;314.2 314.2 314.2;1.019 -0.1826 -1.753]  nHarmo=1  Measurements=None  Decoupling=off  VsMag0=0  VrMag0=0  VsAngle0=0  VrAngle0=0  IsMag0=0  IrMag0=0  IsAngle0=0  IrAngle0=0
      settings: SourceProductBaseCode=PS
  Load {171,894,8468,8478} (4 alike) : spsThreePhaseSeriesRLCLoadLib/Three-Phase Series RLC Load  LConnTagsString=A|B|C  Configuration=Delta  NominalVoltage=10000  Vabc=[1e3 1e3 1e3]  Vabcp=[1e3 1e3 1e3]  NominalFrequency=50  UnbalancedPower=off  ActivePower=9273.6  InductivePower=4491.409  CapacitivePower=0  Pabc=[10e3 9e3 11e3]  QLabc=[100 90 110]  QCabc=[100 90 110]  Pabcp=[10e3 9e3 11e3]  QLabcp=[100 90 110]  QCabcp=[100 90 110]  Measurements=None  LoadType=constant Z
  Load 174 : spsThreePhaseSeriesRLCLoadLib/Three-Phase Series RLC Load  LConnTagsString=A|B|C  Configuration=Delta  NominalVoltage=10000  Vabc=[1e3 1e3 1e3]  Vabcp=[1e3 1e3 1e3]  NominalFrequency=50  UnbalancedPower=off  ActivePower=20865.6  InductivePower=10105.671  CapacitivePower=0  Pabc=[10e3 9e3 11e3]  QLabc=[100 90 110]  QCabc=[100 90 110]  Pabcp=[10e3 9e3 11e3]  QLabcp=[100 90 110]  QCabcp=[100 90 110]  Measurements=None  LoadType=constant Z
  Load 178 : spsThreePhaseSeriesRLCLoadLib/Three-Phase Series RLC Load  LConnTagsString=A|B|C  Configuration=Delta  NominalVoltage=10000  Vabc=[1e3 1e3 1e3]  Vabcp=[1e3 1e3 1e3]  NominalFrequency=50  UnbalancedPower=off  ActivePower=3477.6  InductivePower=1684.279  CapacitivePower=0  Pabc=[10e3 9e3 11e3]  QLabc=[100 90 110]  QCabc=[100 90 110]  Pabcp=[10e3 9e3 11e3]  QLabcp=[100 90 110]  QCabcp=[100 90 110]  Measurements=None  LoadType=constant Z
  Load 1873 : spsThreePhaseSeriesRLCLoadLib/Three-Phase Series RLC Load  LConnTagsString=A|B|C  Configuration=Delta  NominalVoltage=10000  Vabc=[1e3 1e3 1e3]  Vabcp=[1e3 1e3 1e3]  NominalFrequency=50  UnbalancedPower=off  ActivePower=5796  InductivePower=2807.131  CapacitivePower=0  Pabc=[10e3 9e3 11e3]  QLabc=[100 90 110]  QCabc=[100 90 110]  Pabcp=[10e3 9e3 11e3]  QLabcp=[100 90 110]  QCabcp=[100 90 110]  Measurements=None  LoadType=constant Z
  Load 534 : spsThreePhaseSeriesRLCLoadLib/Three-Phase Series RLC Load  LConnTagsString=A|B|C  Configuration=Delta  NominalVoltage=10000  Vabc=[1e3 1e3 1e3]  Vabcp=[1e3 1e3 1e3]  NominalFrequency=50  UnbalancedPower=off  ActivePower=36514.8  InductivePower=17684.925  CapacitivePower=0  Pabc=[10e3 9e3 11e3]  QLabc=[100 90 110]  QCabc=[100 90 110]  Pabcp=[10e3 9e3 11e3]  QLabcp=[100 90 110]  QCabcp=[100 90 110]  Measurements=None  LoadType=constant Z
  Load 535 : spsThreePhaseSeriesRLCLoadLib/Three-Phase Series RLC Load  LConnTagsString=A|B|C  Configuration=Delta  NominalVoltage=10000  Vabc=[1e3 1e3 1e3]  Vabcp=[1e3 1e3 1e3]  NominalFrequency=50  UnbalancedPower=off  ActivePower=18547.2  InductivePower=8982.819  CapacitivePower=0  Pabc=[10e3 9e3 11e3]  QLabc=[100 90 110]  QCabc=[100 90 110]  Pabcp=[10e3 9e3 11e3]  QLabcp=[100 90 110]  QCabcp=[100 90 110]  Measurements=None  LoadType=constant Z
  Load 8042 : spsThreePhaseSeriesRLCLoadLib/Three-Phase Series RLC Load  LConnTagsString=A|B|C  Configuration=Delta  NominalVoltage=10000  Vabc=[1e3 1e3 1e3]  Vabcp=[1e3 1e3 1e3]  NominalFrequency=50  UnbalancedPower=off  ActivePower=1449  InductivePower=701.783  CapacitivePower=0  Pabc=[10e3 9e3 11e3]  QLabc=[100 90 110]  QCabc=[100 90 110]  Pabcp=[10e3 9e3 11e3]  QLabcp=[100 90 110]  QCabcp=[100 90 110]  Measurements=None  LoadType=constant Z
  Load {8130,8193,8201..8202} (4 alike) : spsThreePhaseSeriesRLCLoadLib/Three-Phase Series RLC Load  LConnTagsString=A|B|C  Configuration=Delta  NominalVoltage=10000  Vabc=[1e3 1e3 1e3]  Vabcp=[1e3 1e3 1e3]  NominalFrequency=50  UnbalancedPower=off  ActivePower=23184  InductivePower=11228.524  CapacitivePower=0  Pabc=[10e3 9e3 11e3]  QLabc=[100 90 110]  QCabc=[100 90 110]  Pabcp=[10e3 9e3 11e3]  QLabcp=[100 90 110]  QCabcp=[100 90 110]  Measurements=None  LoadType=constant Z
  Load 8131 : spsThreePhaseSeriesRLCLoadLib/Three-Phase Series RLC Load  LConnTagsString=A|B|C  Configuration=Delta  NominalVoltage=10000  Vabc=[1e3 1e3 1e3]  Vabcp=[1e3 1e3 1e3]  NominalFrequency=50  UnbalancedPower=off  ActivePower=46368  InductivePower=22457.047  CapacitivePower=0  Pabc=[10e3 9e3 11e3]  QLabc=[100 90 110]  QCabc=[100 90 110]  Pabcp=[10e3 9e3 11e3]  QLabcp=[100 90 110]  QCabcp=[100 90 110]  Measurements=None  LoadType=constant Z
  Load 8429 : spsThreePhaseSeriesRLCLoadLib/Three-Phase Series RLC Load  LConnTagsString=A|B|C  Configuration=Delta  NominalVoltage=10000  Vabc=[1e3 1e3 1e3]  Vabcp=[1e3 1e3 1e3]  NominalFrequency=50  UnbalancedPower=off  ActivePower=14490  InductivePower=7017.827  CapacitivePower=0  Pabc=[10e3 9e3 11e3]  QLabc=[100 90 110]  QCabc=[100 90 110]  Pabcp=[10e3 9e3 11e3]  QLabcp=[100 90 110]  QCabcp=[100 90 110]  Measurements=None  LoadType=constant Z
  Load 8590 : spsThreePhaseSeriesRLCLoadLib/Three-Phase Series RLC Load  LConnTagsString=A|B|C  Configuration=Delta  NominalVoltage=10000  Vabc=[1e3 1e3 1e3]  Vabcp=[1e3 1e3 1e3]  NominalFrequency=50  UnbalancedPower=off  ActivePower=5796  InductivePower=2807.131  CapacitivePower=0  Pabc=[10e3 9e3 11e3]  QLabc=[100 90 110]  QCabc=[100 90 110]  Pabcp=[10e3 9e3 11e3]  QLabcp=[100 90 110]  QCabcp=[100 90 110]  Measurements=None  LoadType=constant Z
  Load 8624 : spsThreePhaseSeriesRLCLoadLib/Three-Phase Series RLC Load  LConnTagsString=A|B|C  Configuration=Delta  NominalVoltage=10000  Vabc=[1e3 1e3 1e3]  Vabcp=[1e3 1e3 1e3]  NominalFrequency=50  UnbalancedPower=off  ActivePower=14490  InductivePower=7017.827  CapacitivePower=0  Pabc=[10e3 9e3 11e3]  QLabc=[100 90 110]  QCabc=[100 90 110]  Pabcp=[10e3 9e3 11e3]  QLabcp=[100 90 110]  QCabcp=[100 90 110]  Measurements=None  LoadType=constant Z
  Load 8693 : spsThreePhaseSeriesRLCLoadLib/Three-Phase Series RLC Load  LConnTagsString=A|B|C  Configuration=Delta  NominalVoltage=10000  Vabc=[1e3 1e3 1e3]  Vabcp=[1e3 1e3 1e3]  NominalFrequency=50  UnbalancedPower=off  ActivePower=28980  InductivePower=14035.655  CapacitivePower=0  Pabc=[10e3 9e3 11e3]  QLabc=[100 90 110]  QCabc=[100 90 110]  Pabcp=[10e3 9e3 11e3]  QLabcp=[100 90 110]  QCabcp=[100 90 110]  Measurements=None  LoadType=constant Z
  Load 895 : spsThreePhaseSeriesRLCLoadLib/Three-Phase Series RLC Load  LConnTagsString=A|B|C  Configuration=Delta  NominalVoltage=10000  Vabc=[1e3 1e3 1e3]  Vabcp=[1e3 1e3 1e3]  NominalFrequency=50  UnbalancedPower=off  ActivePower=2318.4  InductivePower=1122.852  CapacitivePower=0  Pabc=[10e3 9e3 11e3]  QLabc=[100 90 110]  QCabc=[100 90 110]  Pabcp=[10e3 9e3 11e3]  QLabcp=[100 90 110]  QCabcp=[100 90 110]  Measurements=None  LoadType=constant Z
  R1 : spsThreePhaseVIMeasurementLib/Three-Phase V-I Measurement  VoltageMeasurement=phase-to-ground  SetLabelV=off  LabelV=Vabc  Vpu=off  VpuLL=off  CurrentMeasurement=yes  SetLabelI=off  LabelI=Iabc  Ipu=off  Pbase=100e6  Vbase=500e3  OutputType=Complex  PhasorSimulation=on  PSBequivalent=0
  R4 : spsThreePhaseVIMeasurementLib/Three-Phase V-I Measurement  VoltageMeasurement=phase-to-ground  SetLabelV=off  LabelV=Vabc  Vpu=off  VpuLL=off  CurrentMeasurement=yes  SetLabelI=off  LabelI=Iabc  Ipu=off  Pbase=100e6  Vbase=500e3  OutputType=Complex  PhasorSimulation=on  PSBequivalent=0
  R6 : spsThreePhaseVIMeasurementLib/Three-Phase V-I Measurement  VoltageMeasurement=phase-to-ground  SetLabelV=off  LabelV=Vabc  Vpu=off  VpuLL=off  CurrentMeasurement=yes  SetLabelI=off  LabelI=Iabc  Ipu=off  Pbase=100e6  Vbase=500e3  OutputType=Complex  PhasorSimulation=on  PSBequivalent=0
  Scope R1 : Scope  NumInputPorts=2
  Scope R4 : Scope  NumInputPorts=2
  Scope R6 : Scope  NumInputPorts=2
  Source PC1_TT2 : spsThreePhaseSourceLib/Three-Phase Source  InternalConnection=Yn  VoltagePhases=off  Voltage=10000  PhaseAngle=0  Voltage_phases=[25e3 25e3 25e3]/sqrt(3)  PhaseAngles_phases=[0 -120 +120]  Frequency=50  NonIdealSource=on  SpecifyImpedance=off  Resistance=0.14  Inductance=0.0031831  ShortCircuitLevel=100e6  BaseVoltage=25e3  XRratio=7  BusType=swing  Pref=10e3  Qref=0  Prefabc=[10e3, 10e3, 10e3]  Qrefabc=[0, 0, 0]  Qmin=-inf  Qmax=inf
  Source Zn : spsSeriesRLCBranchLib/Series RLC Branch  LConnTagsString=__new0  RConnTagsString=__new0  BranchType=RL  Resistance=0.001  Inductance=3.1831e-06  SetiL0=off  InitialCurrent=0  Capacitance=0  Setx0=off  InitialVoltage=0  Measurements=None
  powergui : spspowerguiLib/powergui  Priority=1  SimulationMode=Phasor  SampleTime=50e-6  frequency=50  Iterations=50  frequencyindice=50  Pbase=100e6  ErrMax=1e-4  UnitsV=kV  UnitsW=MW  buscounter=0  FunctionMessages=off  echomessages=off  EnableUseOfTLC=off  CurrentSourceSwitches=off  DisableSnubberDevices=off  DisableRonSwitches=off  DisableVfSwitches=off  DisplayEquations=off  AutomaticDiscreteSolvers=off  SolverType=Tustin/Backward Euler (TBE)  Interpol=off  ExternalGateDelay=off  methode=off  Ts=10  x0status=blocks  SPID=off  SwTol=0  HookPort=off  NonlinearTolerance=1e-4  nMaxIteration=100  ContinueOnMaxIteration=off  RestoreLinks=warning  ResistiveCurrentMeasurement=off  Frange=[0:2:500]  Ylog=off  Xlog=on  ShowGrid=off  save=off  variable=ZData  structure=0  ZoomFFT=off  StartTime=0.0  cycles=1  DisplayStyle=1  fundamental=60  FreqAxis=off  MaxFrequency=1000  frequencyindicesteady=1  RmsSteady=1  display=off
  wires:
  R6/1 -> Scope R6/1
  R6/2 -> Scope R6/2
  R4/1 -> Scope R4/1
  R4/2 -> Scope R4/2
  R1/1 -> Scope R1/1
  R1/2 -> Scope R1/2
  connections:
  Source Zn/RConn1 -- Source PC1_TT2/LConn1
  Source Zn/LConn1 -- Ground/LConn1
  Load 534/LConn1 -- Line 5/RConn1
  Load 534/LConn2 -- Line 5/RConn2
  Load 534/LConn3 -- Line 5/RConn3
  Load 535/LConn1 -- Line 7/RConn1
  Load 535/LConn2 -- Line 7/RConn2
  Load 535/LConn3 -- Line 7/RConn3
  Line 7/LConn1 -- Line 6/RConn1
  Line 7/LConn2 -- Line 6/RConn2
  Line 7/LConn3 -- Line 6/RConn3
  Line 4/RConn1 -- Line 5/LConn1 -- Line 6/LConn1
  Line 4/RConn2 -- Line 5/LConn2 -- Line 6/LConn2
  Line 4/RConn3 -- Line 5/LConn3 -- Line 6/LConn3
  Load 1873/LConn1 -- Line 9/RConn1
  Load 1873/LConn2 -- Line 9/RConn2
  Load 1873/LConn3 -- Line 9/RConn3
  Load 174/LConn1 -- Line 11/RConn1
  Load 174/LConn2 -- Line 11/RConn2
  Load 174/LConn3 -- Line 11/RConn3
  Load 894/LConn1 -- Line 13/RConn1
  Load 894/LConn2 -- Line 13/RConn2
  Load 894/LConn3 -- Line 13/RConn3
  Load 895/LConn1 -- Line 14/RConn1
  Load 895/LConn2 -- Line 14/RConn2
  Load 895/LConn3 -- Line 14/RConn3
  Line 12/RConn1 -- Line 13/LConn1 -- Line 14/LConn1
  Line 12/RConn2 -- Line 13/LConn2 -- Line 14/LConn2
  Line 12/RConn3 -- Line 13/LConn3 -- Line 14/LConn3
  Line 10/RConn1 -- Line 11/LConn1 -- Line 12/LConn1
  Line 10/RConn2 -- Line 11/LConn2 -- Line 12/LConn2
  Line 10/RConn3 -- Line 11/LConn3 -- Line 12/LConn3
  Load 8042/LConn1 -- Line 16/RConn1
  Load 8042/LConn2 -- Line 16/RConn2
  Load 8042/LConn3 -- Line 16/RConn3
  Load 8590/LConn1 -- Line 28/RConn1
  Load 8590/LConn2 -- Line 28/RConn2
  Load 8590/LConn3 -- Line 28/RConn3
  Load 171/LConn1 -- Line 30/RConn1
  Load 171/LConn2 -- Line 30/RConn2
  Load 171/LConn3 -- Line 30/RConn3
  Load 8468/LConn1 -- Line 32/RConn1
  Load 8468/LConn2 -- Line 32/RConn2
  Load 8468/LConn3 -- Line 32/RConn3
  R6/LConn1 -- Line 33/RConn1
  R6/LConn2 -- Line 33/RConn2
  R6/LConn3 -- Line 33/RConn3
  Line 31/RConn1 -- Line 32/LConn1 -- Line 33/LConn1
  Line 31/RConn2 -- Line 32/LConn2 -- Line 33/LConn2
  Line 31/RConn3 -- Line 32/LConn3 -- Line 33/LConn3
  Line 29/RConn1 -- Line 30/LConn1 -- Line 31/LConn1 -- Load 8193/LConn1
  Line 29/RConn2 -- Line 30/LConn2 -- Line 31/LConn2 -- Load 8193/LConn2
  Line 29/RConn3 -- Line 30/LConn3 -- Line 31/LConn3 -- Load 8193/LConn3
  Line 27/RConn1 -- Line 28/LConn1 -- Line 29/LConn1
  Line 27/RConn2 -- Line 28/LConn2 -- Line 29/LConn2
  Line 27/RConn3 -- Line 28/LConn3 -- Line 29/LConn3
  Line 27/LConn1 -- Line 26/RConn1
  Line 27/LConn2 -- Line 26/RConn2
  Line 27/LConn3 -- Line 26/RConn3
  Line 25/RConn1 -- Line 26/LConn1 -- Load 8202/LConn1
  Line 25/RConn2 -- Line 26/LConn2 -- Load 8202/LConn2
  Line 25/RConn3 -- Line 26/LConn3 -- Load 8202/LConn3
  Line 25/LConn1 -- Line 24/RConn1
  Line 25/LConn2 -- Line 24/RConn2
  Line 25/LConn3 -- Line 24/RConn3
  Line 24/LConn1 -- Line 23/RConn1
  Line 24/LConn2 -- Line 23/RConn2
  Line 24/LConn3 -- Line 23/RConn3
  Line 22/RConn1 -- Line 23/LConn1 -- Load 8624/LConn1
  Line 22/RConn2 -- Line 23/LConn2 -- Load 8624/LConn2
  Line 22/RConn3 -- Line 23/LConn3 -- Load 8624/LConn3
  Line 22/LConn1 -- Line 21/RConn1
  Line 22/LConn2 -- Line 21/RConn2
  Line 22/LConn3 -- Line 21/RConn3
  Line 21/LConn1 -- Line 20/RConn1
  Line 21/LConn2 -- Line 20/RConn2
  Line 21/LConn3 -- Line 20/RConn3
  Line 19/RConn1 -- Line 20/LConn1 -- Load 8429/LConn1
  Line 19/RConn2 -- Line 20/LConn2 -- Load 8429/LConn2
  Line 19/RConn3 -- Line 20/LConn3 -- Load 8429/LConn3
  Line 19/LConn1 -- Line 18/RConn1
  Line 19/LConn2 -- Line 18/RConn2
  Line 19/LConn3 -- Line 18/RConn3
  Load 8478/LConn1 -- Line 37/RConn1
  Load 8478/LConn2 -- Line 37/RConn2
  Load 8478/LConn3 -- Line 37/RConn3
  Load 8130/LConn1 -- Line 40/RConn1
  Load 8130/LConn2 -- Line 40/RConn2
  Load 8130/LConn3 -- Line 40/RConn3
  Load 8201/LConn1 -- Line 42/RConn1
  Load 8201/LConn2 -- Line 42/RConn2
  Load 8201/LConn3 -- Line 42/RConn3
  Load 8693/LConn1 -- Line 43/RConn1
  Load 8693/LConn2 -- Line 43/RConn2
  Load 8693/LConn3 -- Line 43/RConn3
  Line 41/RConn1 -- Line 42/LConn1 -- Line 43/LConn1
  Line 41/RConn2 -- Line 42/LConn2 -- Line 43/LConn2
  Line 41/RConn3 -- Line 42/LConn3 -- Line 43/LConn3
  Line 39/RConn1 -- Line 40/LConn1 -- Line 41/LConn1
  Line 39/RConn2 -- Line 40/LConn2 -- Line 41/LConn2
  Line 39/RConn3 -- Line 40/LConn3 -- Line 41/LConn3
  Line 38/RConn1 -- Line 39/LConn1 -- Line im2/LConn1
  Line 38/RConn2 -- Line 39/LConn2 -- Line im2/LConn2
  Line 38/RConn3 -- Line 39/LConn3 -- Line im2/LConn3
  Line 36/RConn1 -- Line 37/LConn1 -- Line 38/LConn1
  Line 36/RConn2 -- Line 37/LConn2 -- Line 38/LConn2
  Line 36/RConn3 -- Line 37/LConn3 -- Line 38/LConn3
  Line 36/LConn1 -- Line 35/RConn1
  Line 36/LConn2 -- Line 35/RConn2
  Line 36/LConn3 -- Line 35/RConn3
  Line im1/RConn1 -- Line 35/LConn1 -- Load 8131/LConn1
  Line im1/RConn2 -- Line 35/LConn2 -- Load 8131/LConn2
  Line im1/RConn3 -- Line 35/LConn3 -- Load 8131/LConn3
  R4/LConn1 -- Line 34/RConn1
  R4/LConn2 -- Line 34/RConn2
  R4/LConn3 -- Line 34/RConn3
  Line im1/LConn1 -- R4/RConn1
  Line im1/LConn2 -- R4/RConn2
  Line im1/LConn3 -- R4/RConn3
  Line 17/RConn1 -- Line 18/LConn1 -- Line 34/LConn1
  Line 17/RConn2 -- Line 18/LConn2 -- Line 34/LConn2
  Line 17/RConn3 -- Line 18/LConn3 -- Line 34/LConn3
  Line 15/RConn1 -- Line 16/LConn1 -- Line 17/LConn1
  Line 15/RConn2 -- Line 16/LConn2 -- Line 17/LConn2
  Line 15/RConn3 -- Line 16/LConn3 -- Line 17/LConn3
  Line 8/RConn1 -- Line 9/LConn1 -- Line 10/LConn1 -- Line 15/LConn1
  Line 8/RConn2 -- Line 9/LConn2 -- Line 10/LConn2 -- Line 15/LConn2
  Line 8/RConn3 -- Line 9/LConn3 -- Line 10/LConn3 -- Line 15/LConn3
  Line 3/RConn1 -- Line 4/LConn1 -- Line 8/LConn1
  Line 3/RConn2 -- Line 4/LConn2 -- Line 8/LConn2
  Line 3/RConn3 -- Line 4/LConn3 -- Line 8/LConn3
  Line 2/RConn1 -- Line 3/LConn1 -- Load 178/LConn1
  Line 2/RConn2 -- Line 3/LConn2 -- Load 178/LConn2
  Line 2/RConn3 -- Line 3/LConn3 -- Load 178/LConn3
  R1/LConn1 -- Line 1/RConn1
  R1/LConn2 -- Line 1/RConn2
  R1/LConn3 -- Line 1/RConn3
  Line 2/LConn1 -- R1/RConn1
  Line 2/LConn2 -- R1/RConn2
  Line 2/LConn3 -- R1/RConn3
  Line 1/LConn1 -- Source PC1_TT2/RConn1
  Line 1/LConn2 -- Source PC1_TT2/RConn2
  Line 1/LConn3 -- Source PC1_TT2/RConn3
